simulink library "outp"  (R2021b)
(part 8 of 11)

      link override Signal_Override/_ovrdflg: Value=KOUTP_FDAGSCmd_enum_ovrdflg
      link override Signal_Override/_ovrdval: Value=KOUTP_FDAGSCmd_enum_ovrdval
  VTHC_FDBlowerCmd_pct_Inproc : FVT_lib/outp/OverrideAndLimit  SystemSampleTime=-1  VariantActivationTime=update diagram  Latency=0  AutoFrameSizeCalculation=off
      link override Signal_Limit/_maxval: Value=KOUTP_FDBlowerCmd_pct_maxval
      link override Signal_Limit/_minval: Value=KOUTP_FDBlowerCmd_pct_minval
      link override Signal_Override/_ovrdflg: Value=KOUTP_FDBlowerCmd_pct_ovrdflg
      link override Signal_Override/_ovrdval: Value=KOUTP_FDBlowerCmd_pct_ovrdval
  VTHC_FDCFGSAirIntCmd_enum_Inproc : FVT_lib/outp/OverrideAndLimit  SystemSampleTime=-1  VariantActivationTime=update diagram  Latency=0  AutoFrameSizeCalculation=off
      link override Signal_Limit/_maxval: Value=KOUTP_FDCFGSAirIntCmd_enum_maxval
      link override Signal_Limit/_minval: Value=KOUTP_FDCFGSAirIntCmd_enum_minval
      link override Signal_Override/_ovrdflg: Value=KOUTP_FDCFGSAirIntCmd_enum_ovrdflg
      link override Signal_Override/_ovrdval: Value=KOUTP_FDCFGSAirIntCmd_enum_ovrdval
  VTHC_FDCFGSAirIntStaSet123_enum_Inproc : FVT_lib/outp/OverrideAndLimit  SystemSampleTime=-1  VariantActivationTime=update diagram  Latency=0  AutoFrameSizeCalculation=off
      link override Signal_Limit/_maxval: Value=KOUTP_FDCFGSAirIntStaSet123_enum_maxval
      link override Signal_Limit/_minval: Value=KOUTP_FDCFGSAirIntStaSet123_enum_minval
      link override Signal_Override/_ovrdflg: Value=KOUTP_FDCFGSAirIntStaSet123_enum_ovrdflg
      link override Signal_Override/_ovrdval: Value=KOUTP_FDCFGSAirIntStaSet123_enum_ovrdval
  VTHC_FDCFGSAirIntStaSet457_enum_Inproc : FVT_lib/outp/OverrideAndLimit  SystemSampleTime=-1  VariantActivationTime=update diagram  Latency=0  AutoFrameSizeCalculation=off
      link override Signal_Limit/_maxval: Value=KOUTP_FDCFGSAirIntStaSet457_enum_maxval
      link override Signal_Limit/_minval: Value=KOUTP_FDCFGSAirIntStaSet457_enum_minval
      link override Signal_Override/_ovrdflg: Value=KOUTP_FDCFGSAirIntStaSet457_enum_ovrdflg
      link override Signal_Override/_ovrdval: Value=KOUTP_FDCFGSAirIntStaSet457_enum_ovrdval
  VTHC_FDCFGSAirIntSta_enum_Inproc : FVT_lib/outp/OverrideAndLimit  SystemSampleTime=-1  VariantActivationTime=update diagram  Latency=0  AutoFrameSizeCalculation=off
      link override Signal_Limit/_maxval: Value=KOUTP_FDCFGSAirIntSta_enum_maxval
      link override Signal_Limit/_minval: Value=KOUTP_FDCFGSAirIntSta_enum_minval
      link override Signal_Override/_ovrdflg: Value=KOUTP_FDCFGSAirIntSta_enum_ovrdflg
      link override Signal_Override/_ovrdval: Value=KOUTP_FDCFGSAirIntSta_enum_ovrdval
  VTHC_FDCFGSChCmd_enum_Inproc : FVT_lib/outp/OverrideAndLimit  SystemSampleTime=-1  VariantActivationTime=update diagram  Latency=0  AutoFrameSizeCalculation=off
      link override Signal_Limit/_maxval: Value=KOUTP_FDCFGSChCmd_enum_maxval
      link override Signal_Limit/_minval: Value=KOUTP_FDCFGSChCmd_enum_minval
      link override Signal_Override/_ovrdflg: Value=KOUTP_FDCFGSChCmd_enum_ovrdflg
      link override Signal_Override/_ovrdval: Value=KOUTP_FDCFGSChCmd_enum_ovrdval
  VTHC_FDCFGSChStaSet123_enum_Inproc : FVT_lib/outp/OverrideAndLimit  SystemSampleTime=-1  VariantActivationTime=update diagram  Latency=0  AutoFrameSizeCalculation=off
      link override Signal_Limit/_maxval: Value=KOUTP_FDCFGSChStaSet123_enum_maxval
      link override Signal_Limit/_minval: Value=KOUTP_FDCFGSChStaSet123_enum_minval
      link override Signal_Override/_ovrdflg: Value=KOUTP_FDCFGSChStaSet123_enum_ovrdflg
      link override Signal_Override/_ovrdval: Value=KOUTP_FDCFGSChStaSet123_enum_ovrdval
  VTHC_FDCFGSChStaSet457_enum_Inproc : FVT_lib/outp/OverrideAndLimit  SystemSampleTime=-1  VariantActivationTime=update diagram  Latency=0  AutoFrameSizeCalculation=off
      link override Signal_Limit/_maxval: Value=KOUTP_FDCFGSChStaSet457_enum_maxval
      link override Signal_Limit/_minval: Value=KOUTP_FDCFGSChStaSet457_enum_minval
      link override Signal_Override/_ovrdflg: Value=KOUTP_FDCFGSChStaSet457_enum_ovrdflg
      link override Signal_Override/_ovrdval: Value=KOUTP_FDCFGSChStaSet457_enum_ovrdval
  VTHC_FDCFGSChSta_enum_Inproc : FVT_lib/outp/OverrideAndLimit  SystemSampleTime=-1  VariantActivationTime=update diagram  Latency=0  AutoFrameSizeCalculation=off
      link override Signal_Limit/_maxval: Value=KOUTP_FDCFGSChSta_enum_maxval
      link override Signal_Limit/_minval: Value=KOUTP_FDCFGSChSta_enum_minval
      link override Signal_Override/_ovrdflg: Value=KOUTP_FDCFGSChSta_enum_ovrdflg
      link override Signal_Override/_ovrdval: Value=KOUTP_FDCFGSChSta_enum_ovrdval
  VTHC_FDCFGSFuncSta_enum_Inproc : FVT_lib/outp/OverrideAndLimit  SystemSampleTime=-1  VariantActivationTime=update diagram  Latency=0  AutoFrameSizeCalculation=off
      link override Signal_Limit/_maxval: Value=KOUTP_FDCFGSFuncSta_enum_maxval
      link override Signal_Limit/_minval: Value=KOUTP_FDCFGSFuncSta_enum_minval
      link override Signal_Override/_ovrdflg: Value=KOUTP_FDCFGSFuncSta_enum_ovrdflg
      link override Signal_Override/_ovrdval: Value=KOUTP_FDCFGSFuncSta_enum_ovrdval
  VTHC_FDCFGSFuncSta_flg_Inproc : FVT_lib/outp/OverrideAndLimit  SystemSampleTime=-1  VariantActivationTime=update diagram  Latency=0  AutoFrameSizeCalculation=off
      link override Signal_Limit/_maxval: Value=KOUTP_FDCFGSFuncSta_flg_maxval
      link override Signal_Limit/_minval: Value=KOUTP_FDCFGSFuncSta_flg_minval
      link override Signal_Override/_ovrdflg: Value=KOUTP_FDCFGSFuncSta_flg_ovrdflg
      link override Signal_Override/_ovrdval: Value=KOUTP_FDCFGSFuncSta_flg_ovrdval
  VTHC_FDCFGSIONCmd_flg_Inproc : FVT_lib/outp/OverrideAndLimit  SystemSampleTime=-1  VariantActivationTime=update diagram  Latency=0  AutoFrameSizeCalculation=off
      link override Signal_Limit/_maxval: Value=KOUTP_FDCFGSIONCmd_flg_maxval
      link override Signal_Limit/_minval: Value=KOUTP_FDCFGSIONCmd_flg_minval
      link override Signal_Override/_ovrdflg: Value=KOUTP_FDCFGSIONCmd_flg_ovrdflg
      link override Signal_Override/_ovrdval: Value=KOUTP_FDCFGSIONCmd_flg_ovrdval
  VTHC_FDCFGSIONSWSta_flg_Inproc : FVT_lib/outp/OverrideAndLimit  SystemSampleTime=-1  VariantActivationTime=update diagram  Latency=0  AutoFrameSizeCalculation=off
      link override Signal_Limit/_maxval: Value=KOUTP_FDCFGSIONSWSta_flg_maxval
      link override Signal_Limit/_minval: Value=KOUTP_FDCFGSIONSWSta_flg_minval
      link override Signal_Override/_ovrdflg: Value=KOUTP_FDCFGSIONSWSta_flg_ovrdflg
      link override Signal_Override/_ovrdval: Value=KOUTP_FDCFGSIONSWSta_flg_ovrdval
  VTHC_FDCFGSLearnCmd_enum_Inproc : FVT_lib/outp/OverrideAndLimit  SystemSampleTime=-1  VariantActivationTime=update diagram  Latency=0  AutoFrameSizeCalculation=off
      link override Signal_Limit/_maxval: Value=KOUTP_FDCFGSLearnCmd_enum_maxval
      link override Signal_Limit/_minval: Value=KOUTP_FDCFGSLearnCmd_enum_minval
      link override Signal_Override/_ovrdflg: Value=KOUTP_FDCFGSLearnCmd_enum_ovrdflg
      link override Signal_Override/_ovrdval: Value=KOUTP_FDCFGSLearnCmd_enum_ovrdval
  VTHC_FDCTHCAirIntZ3Sta_enum_Inproc : FVT_lib/outp/OverrideAndLimit  SystemSampleTime=-1  VariantActivationTime=update diagram  Latency=0  AutoFrameSizeCalculation=off
      link override Signal_Limit/_maxval: Value=KOUTP_FDCTHCAirIntZ3Sta_enum_maxval
      link override Signal_Limit/_minval: Value=KOUTP_FDCTHCAirIntZ3Sta_enum_minval
      link override Signal_Override/_ovrdflg: Value=KOUTP_FDCTHCAirIntZ3Sta_enum_ovrdflg
      link override Signal_Override/_ovrdval: Value=KOUTP_FDCTHCAirIntZ3Sta_enum_ovrdval
  VTHC_FDCTHCCLEVentYStaSet1_enum_Inproc : FVT_lib/outp/OverrideAndLimit  SystemSampleTime=-1  VariantActivationTime=update diagram  Latency=0  AutoFrameSizeCalculation=off
      link override Signal_Limit/_maxval: Value=KOUTP_FDCTHCCLEVentYStaSet1_enum_maxval
      link override Signal_Limit/_minval: Value=KOUTP_FDCTHCCLEVentYStaSet1_enum_minval
      link override Signal_Override/_ovrdflg: Value=KOUTP_FDCTHCCLEVentYStaSet1_enum_ovrdflg
      link override Signal_Override/_ovrdval: Value=KOUTP_FDCTHCCLEVentYStaSet1_enum_ovrdval
  VTHC_FDCTHCCLEVentYStaSet2_enum_Inproc : FVT_lib/outp/OverrideAndLimit  SystemSampleTime=-1  VariantActivationTime=update diagram  Latency=0  AutoFrameSizeCalculation=off
      link override Signal_Limit/_maxval: Value=KOUTP_FDCTHCCLEVentYStaSet2_enum_maxval
      link override Signal_Limit/_minval: Value=KOUTP_FDCTHCCLEVentYStaSet2_enum_minval
      link override Signal_Override/_ovrdflg: Value=KOUTP_FDCTHCCLEVentYStaSet2_enum_ovrdflg
      link override Signal_Override/_ovrdval: Value=KOUTP_FDCTHCCLEVentYStaSet2_enum_ovrdval
  VTHC_FDCTHCCLEVentYStaSet3_enum_Inproc : FVT_lib/outp/OverrideAndLimit  SystemSampleTime=-1  VariantActivationTime=update diagram  Latency=0  AutoFrameSizeCalculation=off
      link override Signal_Limit/_maxval: Value=KOUTP_FDCTHCCLEVentYStaSet3_enum_maxval
      link override Signal_Limit/_minval: Value=KOUTP_FDCTHCCLEVentYStaSet3_enum_minval
      link override Signal_Override/_ovrdflg: Value=KOUTP_FDCTHCCLEVentYStaSet3_enum_ovrdflg
      link override Signal_Override/_ovrdval: Value=KOUTP_FDCTHCCLEVentYStaSet3_enum_ovrdval
  VTHC_FDCTHCCLEVentYStaSet4_enum_Inproc : FVT_lib/outp/OverrideAndLimit  SystemSampleTime=-1  VariantActivationTime=update diagram  Latency=0  AutoFrameSizeCalculation=off
      link override Signal_Limit/_maxval: Value=KOUTP_FDCTHCCLEVentYStaSet4_enum_maxval
      link override Signal_Limit/_minval: Value=KOUTP_FDCTHCCLEVentYStaSet4_enum_minval
      link override Signal_Override/_ovrdflg: Value=KOUTP_FDCTHCCLEVentYStaSet4_enum_ovrdflg
      link override Signal_Override/_ovrdval: Value=KOUTP_FDCTHCCLEVentYStaSet4_enum_ovrdval
  VTHC_FDCTHCCLEVentYStaSet5_enum_Inproc : FVT_lib/outp/OverrideAndLimit  SystemSampleTime=-1  VariantActivationTime=update diagram  Latency=0  AutoFrameSizeCalculation=off
      link override Signal_Limit/_maxval: Value=KOUTP_FDCTHCCLEVentYStaSet5_enum_maxval
      link override Signal_Limit/_minval: Value=KOUTP_FDCTHCCLEVentYStaSet5_enum_minval
      link override Signal_Override/_ovrdflg: Value=KOUTP_FDCTHCCLEVentYStaSet5_enum_ovrdflg
      link override Signal_Override/_ovrdval: Value=KOUTP_FDCTHCCLEVentYStaSet5_enum_ovrdval
  VTHC_FDCTHCCLEVentYStaSet7_enum_Inproc : FVT_lib/outp/OverrideAndLimit  SystemSampleTime=-1  VariantActivationTime=update diagram  Latency=0  AutoFrameSizeCalculation=off
      link override Signal_Limit/_maxval: Value=KOUTP_FDCTHCCLEVentYStaSet7_enum_maxval
      link override Signal_Limit/_minval: Value=KOUTP_FDCTHCCLEVentYStaSet7_enum_minval
      link override Signal_Override/_ovrdflg: Value=KOUTP_FDCTHCCLEVentYStaSet7_enum_ovrdflg
      link override Signal_Override/_ovrdval: Value=KOUTP_FDCTHCCLEVentYStaSet7_enum_ovrdval
  VTHC_FDCTHCCLEVentYSta_enum_Inproc : FVT_lib/outp/OverrideAndLimit  SystemSampleTime=-1  VariantActivationTime=update diagram  Latency=0  AutoFrameSizeCalculation=off
      link override Signal_Limit/_maxval: Value=KOUTP_FDCTHCCLEVentYSta_enum_maxval
      link override Signal_Limit/_minval: Value=KOUTP_FDCTHCCLEVentYSta_enum_minval
      link override Signal_Override/_ovrdflg: Value=KOUTP_FDCTHCCLEVentYSta_enum_ovrdflg
      link override Signal_Override/_ovrdval: Value=KOUTP_FDCTHCCLEVentYSta_enum_ovrdval
  VTHC_FDCTHCCLEVentZStaSet1_enum_Inproc : FVT_lib/outp/OverrideAndLimit  SystemSampleTime=-1  VariantActivationTime=update diagram  Latency=0  AutoFrameSizeCalculation=off
      link override Signal_Limit/_maxval: Value=KOUTP_FDCTHCCLEVentZStaSet1_enum_maxval
      link override Signal_Limit/_minval: Value=KOUTP_FDCTHCCLEVentZStaSet1_enum_minval
      link override Signal_Override/_ovrdflg: Value=KOUTP_FDCTHCCLEVentZStaSet1_enum_ovrdflg
      link override Signal_Override/_ovrdval: Value=KOUTP_FDCTHCCLEVentZStaSet1_enum_ovrdval
  VTHC_FDCTHCCLEVentZStaSet2_enum_Inproc : FVT_lib/outp/OverrideAndLimit  SystemSampleTime=-1  VariantActivationTime=update diagram  Latency=0  AutoFrameSizeCalculation=off
      link override Signal_Limit/_maxval: Value=KOUTP_FDCTHCCLEVentZStaSet2_enum_maxval
      link override Signal_Limit/_minval: Value=KOUTP_FDCTHCCLEVentZStaSet2_enum_minval
      link override Signal_Override/_ovrdflg: Value=KOUTP_FDCTHCCLEVentZStaSet2_enum_ovrdflg
      link override Signal_Override/_ovrdval: Value=KOUTP_FDCTHCCLEVentZStaSet2_enum_ovrdval
  VTHC_FDCTHCCLEVentZStaSet3_enum_Inproc : FVT_lib/outp/OverrideAndLimit  SystemSampleTime=-1  VariantActivationTime=update diagram  Latency=0  AutoFrameSizeCalculation=off
      link override Signal_Limit/_maxval: Value=KOUTP_FDCTHCCLEVentZStaSet3_enum_maxval
      link override Signal_Limit/_minval: Value=KOUTP_FDCTHCCLEVentZStaSet3_enum_minval
      link override Signal_Override/_ovrdflg: Value=KOUTP_FDCTHCCLEVentZStaSet3_enum_ovrdflg
      link override Signal_Override/_ovrdval: Value=KOUTP_FDCTHCCLEVentZStaSet3_enum_ovrdval
  VTHC_FDCTHCCLEVentZStaSet4_enum_Inproc : FVT_lib/outp/OverrideAndLimit  SystemSampleTime=-1  VariantActivationTime=update diagram  Latency=0  AutoFrameSizeCalculation=off
      link override Signal_Limit/_maxval: Value=KOUTP_FDCTHCCLEVentZStaSet4_enum_maxval
      link override Signal_Limit/_minval: Value=KOUTP_FDCTHCCLEVentZStaSet4_enum_minval
      link override Signal_Override/_ovrdflg: Value=KOUTP_FDCTHCCLEVentZStaSet4_enum_ovrdflg
      link override Signal_Override/_ovrdval: Value=KOUTP_FDCTHCCLEVentZStaSet4_enum_ovrdval
  VTHC_FDCTHCCLEVentZStaSet5_enum_Inproc : FVT_lib/outp/OverrideAndLimit  SystemSampleTime=-1  VariantActivationTime=update diagram  Latency=0  AutoFrameSizeCalculation=off
      link override Signal_Limit/_maxval: Value=KOUTP_FDCTHCCLEVentZStaSet5_enum_maxval
      link override Signal_Limit/_minval: Value=KOUTP_FDCTHCCLEVentZStaSet5_enum_minval
      link override Signal_Override/_ovrdflg: Value=KOUTP_FDCTHCCLEVentZStaSet5_enum_ovrdflg
      link override Signal_Override/_ovrdval: Value=KOUTP_FDCTHCCLEVentZStaSet5_enum_ovrdval
  VTHC_FDCTHCCLEVentZStaSet7_enum_Inproc : FVT_lib/outp/OverrideAndLimit  SystemSampleTime=-1  VariantActivationTime=update diagram  Latency=0  AutoFrameSizeCalculation=off
      link override Signal_Limit/_maxval: Value=KOUTP_FDCTHCCLEVentZStaSet7_enum_maxval
      link override Signal_Limit/_minval: Value=KOUTP_FDCTHCCLEVentZStaSet7_enum_minval
      link override Signal_Override/_ovrdflg: Value=KOUTP_FDCTHCCLEVentZStaSet7_enum_ovrdflg
      link override Signal_Override/_ovrdval: Value=KOUTP_FDCTHCCLEVentZStaSet7_enum_ovrdval
  VTHC_FDCTHCCLEVentZSta_enum_Inproc : FVT_lib/outp/OverrideAndLimit  SystemSampleTime=-1  VariantActivationTime=update diagram  Latency=0  AutoFrameSizeCalculation=off
      link override Signal_Limit/_maxval: Value=KOUTP_FDCTHCCLEVentZSta_enum_maxval
      link override Signal_Limit/_minval: Value=KOUTP_FDCTHCCLEVentZSta_enum_minval
      link override Signal_Override/_ovrdflg: Value=KOUTP_FDCTHCCLEVentZSta_enum_ovrdflg
      link override Signal_Override/_ovrdval: Value=KOUTP_FDCTHCCLEVentZSta_enum_ovrdval
  VTHC_FDCTHCCLVentENSta_flg_Inproc : FVT_lib/outp/OverrideAndLimit  SystemSampleTime=-1  VariantActivationTime=update diagram  Latency=0  AutoFrameSizeCalculation=off
      link override Signal_Limit/_maxval: Value=KOUTP_FDCTHCCLVentENSta_flg_maxval
      link override Signal_Limit/_minval: Value=KOUTP_FDCTHCCLVentENSta_flg_minval
      link override Signal_Override/_ovrdflg: Value=KOUTP_FDCTHCCLVentENSta_flg_ovrdflg
      link override Signal_Override/_ovrdval: Value=KOUTP_FDCTHCCLVentENSta_flg_ovrdval
  VTHC_FDCTHCCREVentYStaSet1_enum_Inproc : FVT_lib/outp/OverrideAndLimit  SystemSampleTime=-1  VariantActivationTime=update diagram  Latency=0  AutoFrameSizeCalculation=off
      link override Signal_Limit/_maxval: Value=KOUTP_FDCTHCCREVentYStaSet1_enum_maxval
      link override Signal_Limit/_minval: Value=KOUTP_FDCTHCCREVentYStaSet1_enum_minval
      link override Signal_Override/_ovrdflg: Value=KOUTP_FDCTHCCREVentYStaSet1_enum_ovrdflg
      link override Signal_Override/_ovrdval: Value=KOUTP_FDCTHCCREVentYStaSet1_enum_ovrdval
  VTHC_FDCTHCCREVentYStaSet2_enum_Inproc : FVT_lib/outp/OverrideAndLimit  SystemSampleTime=-1  VariantActivationTime=update diagram  Latency=0  AutoFrameSizeCalculation=off
      link override Signal_Limit/_maxval: Value=KOUTP_FDCTHCCREVentYStaSet2_enum_maxval
      link override Signal_Limit/_minval: Value=KOUTP_FDCTHCCREVentYStaSet2_enum_minval
      link override Signal_Override/_ovrdflg: Value=KOUTP_FDCTHCCREVentYStaSet2_enum_ovrdflg
      link override Signal_Override/_ovrdval: Value=KOUTP_FDCTHCCREVentYStaSet2_enum_ovrdval
  VTHC_FDCTHCCREVentYStaSet3_enum_Inproc : FVT_lib/outp/OverrideAndLimit  SystemSampleTime=-1  VariantActivationTime=update diagram  Latency=0  AutoFrameSizeCalculation=off
      link override Signal_Limit/_maxval: Value=KOUTP_FDCTHCCREVentYStaSet3_enum_maxval
      link override Signal_Limit/_minval: Value=KOUTP_FDCTHCCREVentYStaSet3_enum_minval
      link override Signal_Override/_ovrdflg: Value=KOUTP_FDCTHCCREVentYStaSet3_enum_ovrdflg
      link override Signal_Override/_ovrdval: Value=KOUTP_FDCTHCCREVentYStaSet3_enum_ovrdval
  VTHC_FDCTHCCREVentYStaSet4_enum_Inproc : FVT_lib/outp/OverrideAndLimit  SystemSampleTime=-1  VariantActivationTime=update diagram  Latency=0  AutoFrameSizeCalculation=off
      link override Signal_Limit/_maxval: Value=KOUTP_FDCTHCCREVentYStaSet4_enum_maxval
      link override Signal_Limit/_minval: Value=KOUTP_FDCTHCCREVentYStaSet4_enum_minval
      link override Signal_Override/_ovrdflg: Value=KOUTP_FDCTHCCREVentYStaSet4_enum_ovrdflg
      link override Signal_Override/_ovrdval: Value=KOUTP_FDCTHCCREVentYStaSet4_enum_ovrdval
  VTHC_FDCTHCCREVentYStaSet5_enum_Inproc : FVT_lib/outp/OverrideAndLimit  SystemSampleTime=-1  VariantActivationTime=update diagram  Latency=0  AutoFrameSizeCalculation=off
      link override Signal_Limit/_maxval: Value=KOUTP_FDCTHCCREVentYStaSet5_enum_maxval
      link override Signal_Limit/_minval: Value=KOUTP_FDCTHCCREVentYStaSet5_enum_minval
      link override Signal_Override/_ovrdflg: Value=KOUTP_FDCTHCCREVentYStaSet5_enum_ovrdflg
      link override Signal_Override/_ovrdval: Value=KOUTP_FDCTHCCREVentYStaSet5_enum_ovrdval
  VTHC_FDCTHCCREVentYStaSet7_enum_Inproc : FVT_lib/outp/OverrideAndLimit  SystemSampleTime=-1  VariantActivationTime=update diagram  Latency=0  AutoFrameSizeCalculation=off
      link override Signal_Limit/_maxval: Value=KOUTP_FDCTHCCREVentYStaSet7_enum_maxval
      link override Signal_Limit/_minval: Value=KOUTP_FDCTHCCREVentYStaSet7_enum_minval
      link override Signal_Override/_ovrdflg: Value=KOUTP_FDCTHCCREVentYStaSet7_enum_ovrdflg
      link override Signal_Override/_ovrdval: Value=KOUTP_FDCTHCCREVentYStaSet7_enum_ovrdval
  VTHC_FDCTHCCREVentYSta_enum_Inproc : FVT_lib/outp/OverrideAndLimit  SystemSampleTime=-1  VariantActivationTime=update diagram  Latency=0  AutoFrameSizeCalculation=off
      link override Signal_Limit/_maxval: Value=KOUTP_FDCTHCCREVentYSta_enum_maxval
      link override Signal_Limit/_minval: Value=KOUTP_FDCTHCCREVentYSta_enum_minval
      link override Signal_Override/_ovrdflg: Value=KOUTP_FDCTHCCREVentYSta_enum_ovrdflg
      link override Signal_Override/_ovrdval: Value=KOUTP_FDCTHCCREVentYSta_enum_ovrdval
  VTHC_FDCTHCCREVentZStaSet1_enum_Inproc : FVT_lib/outp/OverrideAndLimit  SystemSampleTime=-1  VariantActivationTime=update diagram  Latency=0  AutoFrameSizeCalculation=off
      link override Signal_Limit/_maxval: Value=KOUTP_FDCTHCCREVentZStaSet1_enum_maxval
      link override Signal_Limit/_minval: Value=KOUTP_FDCTHCCREVentZStaSet1_enum_minval
      link override Signal_Override/_ovrdflg: Value=KOUTP_FDCTHCCREVentZStaSet1_enum_ovrdflg
      link override Signal_Override/_ovrdval: Value=KOUTP_FDCTHCCREVentZStaSet1_enum_ovrdval
  VTHC_FDCTHCCREVentZStaSet2_enum_Inproc : FVT_lib/outp/OverrideAndLimit  SystemSampleTime=-1  VariantActivationTime=update diagram  Latency=0  AutoFrameSizeCalculation=off
      link override Signal_Limit/_maxval: Value=KOUTP_FDCTHCCREVentZStaSet2_enum_maxval
      link override Signal_Limit/_minval: Value=KOUTP_FDCTHCCREVentZStaSet2_enum_minval
      link override Signal_Override/_ovrdflg: Value=KOUTP_FDCTHCCREVentZStaSet2_enum_ovrdflg
      link override Signal_Override/_ovrdval: Value=KOUTP_FDCTHCCREVentZStaSet2_enum_ovrdval
  VTHC_FDCTHCCREVentZStaSet3_enum_Inproc : FVT_lib/outp/OverrideAndLimit  SystemSampleTime=-1  VariantActivationTime=update diagram  Latency=0  AutoFrameSizeCalculation=off
      link override Signal_Limit/_maxval: Value=KOUTP_FDCTHCCREVentZStaSet3_enum_maxval
      link override Signal_Limit/_minval: Value=KOUTP_FDCTHCCREVentZStaSet3_enum_minval
      link override Signal_Override/_ovrdflg: Value=KOUTP_FDCTHCCREVentZStaSet3_enum_ovrdflg
      link override Signal_Override/_ovrdval: Value=KOUTP_FDCTHCCREVentZStaSet3_enum_ovrdval
  VTHC_FDCTHCCREVentZStaSet4_enum_Inproc : FVT_lib/outp/OverrideAndLimit  SystemSampleTime=-1  VariantActivationTime=update diagram  Latency=0  AutoFrameSizeCalculation=off
      link override Signal_Limit/_maxval: Value=KOUTP_FDCTHCCREVentZStaSet4_enum_maxval
      link override Signal_Limit/_minval: Value=KOUTP_FDCTHCCREVentZStaSet4_enum_minval
      link override Signal_Override/_ovrdflg: Value=KOUTP_FDCTHCCREVentZStaSet4_enum_ovrdflg
      link override Signal_Override/_ovrdval: Value=KOUTP_FDCTHCCREVentZStaSet4_enum_ovrdval
  VTHC_FDCTHCCREVentZStaSet5_enum_Inproc : FVT_lib/outp/OverrideAndLimit  SystemSampleTime=-1  VariantActivationTime=update diagram  Latency=0  AutoFrameSizeCalculation=off
      link override Signal_Limit/_maxval: Value=KOUTP_FDCTHCCREVentZStaSet5_enum_maxval
      link override Signal_Limit/_minval: Value=KOUTP_FDCTHCCREVentZStaSet5_enum_minval
      link override Signal_Override/_ovrdflg: Value=KOUTP_FDCTHCCREVentZStaSet5_enum_ovrdflg
      link override Signal_Override/_ovrdval: Value=KOUTP_FDCTHCCREVentZStaSet5_enum_ovrdval
  VTHC_FDCTHCCREVentZStaSet7_enum_Inproc : FVT_lib/outp/OverrideAndLimit  SystemSampleTime=-1  VariantActivationTime=update diagram  Latency=0  AutoFrameSizeCalculation=off
      link override Signal_Limit/_maxval: Value=KOUTP_FDCTHCCREVentZStaSet7_enum_maxval
      link override Signal_Limit/_minval: Value=KOUTP_FDCTHCCREVentZStaSet7_enum_minval
      link override Signal_Override/_ovrdflg: Value=KOUTP_FDCTHCCREVentZStaSet7_enum_ovrdflg
      link override Signal_Override/_ovrdval: Value=KOUTP_FDCTHCCREVentZStaSet7_enum_ovrdval
  VTHC_FDCTHCCREVentZSta_enum_Inproc : FVT_lib/outp/OverrideAndLimit  SystemSampleTime=-1  VariantActivationTime=update diagram  Latency=0  AutoFrameSizeCalculation=off
      link override Signal_Limit/_maxval: Value=KOUTP_FDCTHCCREVentZSta_enum_maxval
      link override Signal_Limit/_minval: Value=KOUTP_FDCTHCCREVentZSta_enum_minval
      link override Signal_Override/_ovrdflg: Value=KOUTP_FDCTHCCREVentZSta_enum_ovrdflg
      link override Signal_Override/_ovrdval: Value=KOUTP_FDCTHCCREVentZSta_enum_ovrdval
  VTHC_FDCTHCCRVentENSta_flg_Inproc : FVT_lib/outp/OverrideAndLimit  SystemSampleTime=-1  VariantActivationTime=update diagram  Latency=0  AutoFrameSizeCalculation=off
      link override Signal_Limit/_maxval: Value=KOUTP_FDCTHCCRVentENSta_flg_maxval
      link override Signal_Limit/_minval: Value=KOUTP_FDCTHCCRVentENSta_flg_minval
      link override Signal_Override/_ovrdflg: Value=KOUTP_FDCTHCCRVentENSta_flg_ovrdflg
      link override Signal_Override/_ovrdval: Value=KOUTP_FDCTHCCRVentENSta_flg_ovrdval
  VTHC_FDCTHCLEVentModeSta_enum_Inproc : FVT_lib/outp/OverrideAndLimit  SystemSampleTime=-1  VariantActivationTime=update diagram  Latency=0  AutoFrameSizeCalculation=off
      link override Signal_Limit/_maxval: Value=KOUTP_FDCTHCLEVentModeSta_enum_maxval
      link override Signal_Limit/_minval: Value=KOUTP_FDCTHCLEVentModeSta_enum_minval
      link override Signal_Override/_ovrdflg: Value=KOUTP_FDCTHCLEVentModeSta_enum_ovrdflg
      link override Signal_Override/_ovrdval: Value=KOUTP_FDCTHCLEVentModeSta_enum_ovrdval
  VTHC_FDCTHCLEVentYStaSet1_enum_Inproc : FVT_lib/outp/OverrideAndLimit  SystemSampleTime=-1  VariantActivationTime=update diagram  Latency=0  AutoFrameSizeCalculation=off
      link override Signal_Limit/_maxval: Value=KOUTP_FDCTHCLEVentYStaSet1_enum_maxval
      link override Signal_Limit/_minval: Value=KOUTP_FDCTHCLEVentYStaSet1_enum_minval
      link override Signal_Override/_ovrdflg: Value=KOUTP_FDCTHCLEVentYStaSet1_enum_ovrdflg
      link override Signal_Override/_ovrdval: Value=KOUTP_FDCTHCLEVentYStaSet1_enum_ovrdval
  VTHC_FDCTHCLEVentYStaSet2_enum_Inproc : FVT_lib/outp/OverrideAndLimit  SystemSampleTime=-1  VariantActivationTime=update diagram  Latency=0  AutoFrameSizeCalculation=off
      link override Signal_Limit/_maxval: Value=KOUTP_FDCTHCLEVentYStaSet2_enum_maxval
      link override Signal_Limit/_minval: Value=KOUTP_FDCTHCLEVentYStaSet2_enum_minval
      link override Signal_Override/_ovrdflg: Value=KOUTP_FDCTHCLEVentYStaSet2_enum_ovrdflg
      link override Signal_Override/_ovrdval: Value=KOUTP_FDCTHCLEVentYStaSet2_enum_ovrdval
  VTHC_FDCTHCLEVentYStaSet3_enum_Inproc : FVT_lib/outp/OverrideAndLimit  SystemSampleTime=-1  VariantActivationTime=update diagram  Latency=0  AutoFrameSizeCalculation=off
      link override Signal_Limit/_maxval: Value=KOUTP_FDCTHCLEVentYStaSet3_enum_maxval
      link override Signal_Limit/_minval: Value=KOUTP_FDCTHCLEVentYStaSet3_enum_minval
      link override Signal_Override/_ovrdflg: Value=KOUTP_FDCTHCLEVentYStaSet3_enum_ovrdflg
      link override Signal_Override/_ovrdval: Value=KOUTP_FDCTHCLEVentYStaSet3_enum_ovrdval
  VTHC_FDCTHCLEVentYStaSet4_enum_Inproc : FVT_lib/outp/OverrideAndLimit  SystemSampleTime=-1  VariantActivationTime=update diagram  Latency=0  AutoFrameSizeCalculation=off
      link override Signal_Limit/_maxval: Value=KOUTP_FDCTHCLEVentYStaSet4_enum_maxval
      link override Signal_Limit/_minval: Value=KOUTP_FDCTHCLEVentYStaSet4_enum_minval
      link override Signal_Override/_ovrdflg: Value=KOUTP_FDCTHCLEVentYStaSet4_enum_ovrdflg
      link override Signal_Override/_ovrdval: Value=KOUTP_FDCTHCLEVentYStaSet4_enum_ovrdval
  VTHC_FDCTHCLEVentYStaSet5_enum_Inproc : FVT_lib/outp/OverrideAndLimit  SystemSampleTime=-1  VariantActivationTime=update diagram  Latency=0  AutoFrameSizeCalculation=off
      link override Signal_Limit/_maxval: Value=KOUTP_FDCTHCLEVentYStaSet5_enum_maxval
      link override Signal_Limit/_minval: Value=KOUTP_FDCTHCLEVentYStaSet5_enum_minval
      link override Signal_Override/_ovrdflg: Value=KOUTP_FDCTHCLEVentYStaSet5_enum_ovrdflg
      link override Signal_Override/_ovrdval: Value=KOUTP_FDCTHCLEVentYStaSet5_enum_ovrdval
  VTHC_FDCTHCLEVentYStaSet7_enum_Inproc : FVT_lib/outp/OverrideAndLimit  SystemSampleTime=-1  VariantActivationTime=update diagram  Latency=0  AutoFrameSizeCalculation=off
      link override Signal_Limit/_maxval: Value=KOUTP_FDCTHCLEVentYStaSet7_enum_maxval
      link override Signal_Limit/_minval: Value=KOUTP_FDCTHCLEVentYStaSet7_enum_minval
      link override Signal_Override/_ovrdflg: Value=KOUTP_FDCTHCLEVentYStaSet7_enum_ovrdflg
      link override Signal_Override/_ovrdval: Value=KOUTP_FDCTHCLEVentYStaSet7_enum_ovrdval
  VTHC_FDCTHCLEVentYSta_enum_Inproc : FVT_lib/outp/OverrideAndLimit  SystemSampleTime=-1  VariantActivationTime=update diagram  Latency=0  AutoFrameSizeCalculation=off
      link override Signal_Limit/_maxval: Value=KOUTP_FDCTHCLEVentYSta_enum_maxval
      link override Signal_Limit/_minval: Value=KOUTP_FDCTHCLEVentYSta_enum_minval
      link override Signal_Override/_ovrdflg: Value=KOUTP_FDCTHCLEVentYSta_enum_ovrdflg
      link override Signal_Override/_ovrdval: Value=KOUTP_FDCTHCLEVentYSta_enum_ovrdval
  VTHC_FDCTHCLEVentZStaSet1_enum_Inproc : FVT_lib/outp/OverrideAndLimit  SystemSampleTime=-1  VariantActivationTime=update diagram  Latency=0  AutoFrameSizeCalculation=off
      link override Signal_Limit/_maxval: Value=KOUTP_FDCTHCLEVentZStaSet1_enum_maxval
      link override Signal_Limit/_minval: Value=KOUTP_FDCTHCLEVentZStaSet1_enum_minval
      link override Signal_Override/_ovrdflg: Value=KOUTP_FDCTHCLEVentZStaSet1_enum_ovrdflg
      link override Signal_Override/_ovrdval: Value=KOUTP_FDCTHCLEVentZStaSet1_enum_ovrdval
  VTHC_FDCTHCLEVentZStaSet2_enum_Inproc : FVT_lib/outp/OverrideAndLimit  SystemSampleTime=-1  VariantActivationTime=update diagram  Latency=0  AutoFrameSizeCalculation=off
      link override Signal_Limit/_maxval: Value=KOUTP_FDCTHCLEVentZStaSet2_enum_maxval
      link override Signal_Limit/_minval: Value=KOUTP_FDCTHCLEVentZStaSet2_enum_minval
      link override Signal_Override/_ovrdflg: Value=KOUTP_FDCTHCLEVentZStaSet2_enum_ovrdflg
      link override Signal_Override/_ovrdval: Value=KOUTP_FDCTHCLEVentZStaSet2_enum_ovrdval
  VTHC_FDCTHCLEVentZStaSet3_enum_Inproc : FVT_lib/outp/OverrideAndLimit  SystemSampleTime=-1  VariantActivationTime=update diagram  Latency=0  AutoFrameSizeCalculation=off
      link override Signal_Limit/_maxval: Value=KOUTP_FDCTHCLEVentZStaSet3_enum_maxval
      link override Signal_Limit/_minval: Value=KOUTP_FDCTHCLEVentZStaSet3_enum_minval
      link override Signal_Override/_ovrdflg: Value=KOUTP_FDCTHCLEVentZStaSet3_enum_ovrdflg
      link override Signal_Override/_ovrdval: Value=KOUTP_FDCTHCLEVentZStaSet3_enum_ovrdval
  VTHC_FDCTHCLEVentZStaSet4_enum_Inproc : FVT_lib/outp/OverrideAndLimit  SystemSampleTime=-1  VariantActivationTime=update diagram  Latency=0  AutoFrameSizeCalculation=off
      link override Signal_Limit/_maxval: Value=KOUTP_FDCTHCLEVentZStaSet4_enum_maxval
      link override Signal_Limit/_minval: Value=KOUTP_FDCTHCLEVentZStaSet4_enum_minval
      link override Signal_Override/_ovrdflg: Value=KOUTP_FDCTHCLEVentZStaSet4_enum_ovrdflg
      link override Signal_Override/_ovrdval: Value=KOUTP_FDCTHCLEVentZStaSet4_enum_ovrdval
  VTHC_FDCTHCLEVentZStaSet5_enum_Inproc : FVT_lib/outp/OverrideAndLimit  SystemSampleTime=-1  VariantActivationTime=update diagram  Latency=0  AutoFrameSizeCalculation=off
      link override Signal_Limit/_maxval: Value=KOUTP_FDCTHCLEVentZStaSet5_enum_maxval
      link override Signal_Limit/_minval: Value=KOUTP_FDCTHCLEVentZStaSet5_enum_minval
      link override Signal_Override/_ovrdflg: Value=KOUTP_FDCTHCLEVentZStaSet5_enum_ovrdflg
      link override Signal_Override/_ovrdval: Value=KOUTP_FDCTHCLEVentZStaSet5_enum_ovrdval
  VTHC_FDCTHCLEVentZStaSet7_enum_Inproc : FVT_lib/outp/OverrideAndLimit  SystemSampleTime=-1  VariantActivationTime=update diagram  Latency=0  AutoFrameSizeCalculation=off
      link override Signal_Limit/_maxval: Value=KOUTP_FDCTHCLEVentZStaSet7_enum_maxval
      link override Signal_Limit/_minval: Value=KOUTP_FDCTHCLEVentZStaSet7_enum_minval
      link override Signal_Override/_ovrdflg: Value=KOUTP_FDCTHCLEVentZStaSet7_enum_ovrdflg
      link override Signal_Override/_ovrdval: Value=KOUTP_FDCTHCLEVentZStaSet7_enum_ovrdval
  VTHC_FDCTHCLEVentZSta_enum_Inproc : FVT_lib/outp/OverrideAndLimit  SystemSampleTime=-1  VariantActivationTime=update diagram  Latency=0  AutoFrameSizeCalculation=off
      link override Signal_Limit/_maxval: Value=KOUTP_FDCTHCLEVentZSta_enum_maxval
      link override Signal_Limit/_minval: Value=KOUTP_FDCTHCLEVentZSta_enum_minval
      link override Signal_Override/_ovrdflg: Value=KOUTP_FDCTHCLEVentZSta_enum_ovrdflg
      link override Signal_Override/_ovrdval: Value=KOUTP_FDCTHCLEVentZSta_enum_ovrdval
  VTHC_FDCTHCLVentENSta_flg_Inproc : FVT_lib/outp/OverrideAndLimit  SystemSampleTime=-1  VariantActivationTime=update diagram  Latency=0  AutoFrameSizeCalculation=off
      link override Signal_Limit/_maxval: Value=KOUTP_FDCTHCLVentENSta_flg_maxval
      link override Signal_Limit/_minval: Value=KOUTP_FDCTHCLVentENSta_flg_minval
      link override Signal_Override/_ovrdflg: Value=KOUTP_FDCTHCLVentENSta_flg_ovrdflg
      link override Signal_Override/_ovrdval: Value=KOUTP_FDCTHCLVentENSta_flg_ovrdval
  VTHC_FDCTHCMAPTCForceOFFSta_flg_Inproc : FVT_lib/outp/OverrideAndLimit  SystemSampleTime=-1  VariantActivationTime=update diagram  Latency=0  AutoFrameSizeCalculation=off
      link override Signal_Limit/_maxval: Value=KOUTP_FDCTHCMAPTCForceOFFSta_flg_maxval
      link override Signal_Limit/_minval: Value=KOUTP_FDCTHCMAPTCForceOFFSta_flg_minval
      link override Signal_Override/_ovrdflg: Value=KOUTP_FDCTHCMAPTCForceOFFSta_flg_ovrdflg
      link override Signal_Override/_ovrdval: Value=KOUTP_FDCTHCMAPTCForceOFFSta_flg_ovrdval
  VTHC_FDCTHCMPreWPTCHeatSta_enum_Inproc : FVT_lib/outp/OverrideAndLimit  SystemSampleTime=-1  VariantActivationTime=update diagram  Latency=0  AutoFrameSizeCalculation=off
      link override Signal_Limit/_maxval: Value=KOUTP_FDCTHCMPreWPTCHeatSta_enum_maxval
      link override Signal_Limit/_minval: Value=KOUTP_FDCTHCMPreWPTCHeatSta_enum_minval
      link override Signal_Override/_ovrdflg: Value=KOUTP_FDCTHCMPreWPTCHeatSta_enum_ovrdflg
      link override Signal_Override/_ovrdval: Value=KOUTP_FDCTHCMPreWPTCHeatSta_enum_ovrdval
  VTHC_FDCTHCREVentModeSta_enum_Inproc : FVT_lib/outp/OverrideAndLimit  SystemSampleTime=-1  VariantActivationTime=update diagram  Latency=0  AutoFrameSizeCalculation=off
      link override Signal_Limit/_maxval: Value=KOUTP_FDCTHCREVentModeSta_enum_maxval
      link override Signal_Limit/_minval: Value=KOUTP_FDCTHCREVentModeSta_enum_minval
      link override Signal_Override/_ovrdflg: Value=KOUTP_FDCTHCREVentModeSta_enum_ovrdflg
      link override Signal_Override/_ovrdval: Value=KOUTP_FDCTHCREVentModeSta_enum_ovrdval
  VTHC_FDCTHCREVentYStaSet1_enum_Inproc : FVT_lib/outp/OverrideAndLimit  SystemSampleTime=-1  VariantActivationTime=update diagram  Latency=0  AutoFrameSizeCalculation=off
      link override Signal_Limit/_maxval: Value=KOUTP_FDCTHCREVentYStaSet1_enum_maxval
      link override Signal_Limit/_minval: Value=KOUTP_FDCTHCREVentYStaSet1_enum_minval
      link override Signal_Override/_ovrdflg: Value=KOUTP_FDCTHCREVentYStaSet1_enum_ovrdflg
      link override Signal_Override/_ovrdval: Value=KOUTP_FDCTHCREVentYStaSet1_enum_ovrdval
  VTHC_FDCTHCREVentYStaSet2_enum_Inproc : FVT_lib/outp/OverrideAndLimit  SystemSampleTime=-1  VariantActivationTime=update diagram  Latency=0  AutoFrameSizeCalculation=off
      link override Signal_Limit/_maxval: Value=KOUTP_FDCTHCREVentYStaSet2_enum_maxval
      link override Signal_Limit/_minval: Value=KOUTP_FDCTHCREVentYStaSet2_enum_minval
      link override Signal_Override/_ovrdflg: Value=KOUTP_FDCTHCREVentYStaSet2_enum_ovrdflg
      link override Signal_Override/_ovrdval: Value=KOUTP_FDCTHCREVentYStaSet2_enum_ovrdval
  VTHC_FDCTHCREVentYStaSet3_enum_Inproc : FVT_lib/outp/OverrideAndLimit  SystemSampleTime=-1  VariantActivationTime=update diagram  Latency=0  AutoFrameSizeCalculation=off
      link override Signal_Limit/_maxval: Value=KOUTP_FDCTHCREVentYStaSet3_enum_maxval
      link override Signal_Limit/_minval: Value=KOUTP_FDCTHCREVentYStaSet3_enum_minval
      link override Signal_Override/_ovrdflg: Value=KOUTP_FDCTHCREVentYStaSet3_enum_ovrdflg
      link override Signal_Override/_ovrdval: Value=KOUTP_FDCTHCREVentYStaSet3_enum_ovrdval
  VTHC_FDCTHCREVentYStaSet4_enum_Inproc : FVT_lib/outp/OverrideAndLimit  SystemSampleTime=-1  VariantActivationTime=update diagram  Latency=0  AutoFrameSizeCalculation=off
      link override Signal_Limit/_maxval: Value=KOUTP_FDCTHCREVentYStaSet4_enum_maxval
      link override Signal_Limit/_minval: Value=KOUTP_FDCTHCREVentYStaSet4_enum_minval
      link override Signal_Override/_ovrdflg: Value=KOUTP_FDCTHCREVentYStaSet4_enum_ovrdflg
      link override Signal_Override/_ovrdval: Value=KOUTP_FDCTHCREVentYStaSet4_enum_ovrdval
  VTHC_FDCTHCREVentYStaSet5_enum_Inproc : FVT_lib/outp/OverrideAndLimit  SystemSampleTime=-1  VariantActivationTime=update diagram  Latency=0  AutoFrameSizeCalculation=off
      link override Signal_Limit/_maxval: Value=KOUTP_FDCTHCREVentYStaSet5_enum_maxval
      link override Signal_Limit/_minval: Value=KOUTP_FDCTHCREVentYStaSet5_enum_minval
      link override Signal_Override/_ovrdflg: Value=KOUTP_FDCTHCREVentYStaSet5_enum_ovrdflg
      link override Signal_Override/_ovrdval: Value=KOUTP_FDCTHCREVentYStaSet5_enum_ovrdval
  VTHC_FDCTHCREVentYStaSet7_enum_Inproc : FVT_lib/outp/OverrideAndLimit  SystemSampleTime=-1  VariantActivationTime=update diagram  Latency=0  AutoFrameSizeCalculation=off
      link override Signal_Limit/_maxval: Value=KOUTP_FDCTHCREVentYStaSet7_enum_maxval
      link override Signal_Limit/_minval: Value=KOUTP_FDCTHCREVentYStaSet7_enum_minval
      link override Signal_Override/_ovrdflg: Value=KOUTP_FDCTHCREVentYStaSet7_enum_ovrdflg
      link override Signal_Override/_ovrdval: Value=KOUTP_FDCTHCREVentYStaSet7_enum_ovrdval
  VTHC_FDCTHCREVentYSta_enum_Inproc : FVT_lib/outp/OverrideAndLimit  SystemSampleTime=-1  VariantActivationTime=update diagram  Latency=0  AutoFrameSizeCalculation=off
      link override Signal_Limit/_maxval: Value=KOUTP_FDCTHCREVentYSta_enum_maxval
      link override Signal_Limit/_minval: Value=KOUTP_FDCTHCREVentYSta_enum_minval
      link override Signal_Override/_ovrdflg: Value=KOUTP_FDCTHCREVentYSta_enum_ovrdflg
      link override Signal_Override/_ovrdval: Value=KOUTP_FDCTHCREVentYSta_enum_ovrdval
  VTHC_FDCTHCREVentZStaSet1_enum_Inproc : FVT_lib/outp/OverrideAndLimit  SystemSampleTime=-1  VariantActivationTime=update diagram  Latency=0  AutoFrameSizeCalculation=off
      link override Signal_Limit/_maxval: Value=KOUTP_FDCTHCREVentZStaSet1_enum_maxval
      link override Signal_Limit/_minval: Value=KOUTP_FDCTHCREVentZStaSet1_enum_minval
      link override Signal_Override/_ovrdflg: Value=KOUTP_FDCTHCREVentZStaSet1_enum_ovrdflg
      link override Signal_Override/_ovrdval: Value=KOUTP_FDCTHCREVentZStaSet1_enum_ovrdval
  VTHC_FDCTHCREVentZStaSet2_enum_Inproc : FVT_lib/outp/OverrideAndLimit  SystemSampleTime=-1  VariantActivationTime=update diagram  Latency=0  AutoFrameSizeCalculation=off
      link override Signal_Limit/_maxval: Value=KOUTP_FDCTHCREVentZStaSet2_enum_maxval
      link override Signal_Limit/_minval: Value=KOUTP_FDCTHCREVentZStaSet2_enum_minval
      link override Signal_Override/_ovrdflg: Value=KOUTP_FDCTHCREVentZStaSet2_enum_ovrdflg
      link override Signal_Override/_ovrdval: Value=KOUTP_FDCTHCREVentZStaSet2_enum_ovrdval
  VTHC_FDCTHCREVentZStaSet3_enum_Inproc : FVT_lib/outp/OverrideAndLimit  SystemSampleTime=-1  VariantActivationTime=update diagram  Latency=0  AutoFrameSizeCalculation=off
      link override Signal_Limit/_maxval: Value=KOUTP_FDCTHCREVentZStaSet3_enum_maxval
      link override Signal_Limit/_minval: Value=KOUTP_FDCTHCREVentZStaSet3_enum_minval
      link override Signal_Override/_ovrdflg: Value=KOUTP_FDCTHCREVentZStaSet3_enum_ovrdflg
      link override Signal_Override/_ovrdval: Value=KOUTP_FDCTHCREVentZStaSet3_enum_ovrdval
  VTHC_FDCTHCREVentZStaSet4_enum_Inproc : FVT_lib/outp/OverrideAndLimit  SystemSampleTime=-1  VariantActivationTime=update diagram  Latency=0  AutoFrameSizeCalculation=off
      link override Signal_Limit/_maxval: Value=KOUTP_FDCTHCREVentZStaSet4_enum_maxval
      link override Signal_Limit/_minval: Value=KOUTP_FDCTHCREVentZStaSet4_enum_minval
      link override Signal_Override/_ovrdflg: Value=KOUTP_FDCTHCREVentZStaSet4_enum_ovrdflg
      link override Signal_Override/_ovrdval: Value=KOUTP_FDCTHCREVentZStaSet4_enum_ovrdval
  VTHC_FDCTHCREVentZStaSet5_enum_Inproc : FVT_lib/outp/OverrideAndLimit  SystemSampleTime=-1  VariantActivationTime=update diagram  Latency=0  AutoFrameSizeCalculation=off
      link override Signal_Limit/_maxval: Value=KOUTP_FDCTHCREVentZStaSet5_enum_maxval
      link override Signal_Limit/_minval: Value=KOUTP_FDCTHCREVentZStaSet5_enum_minval
      link override Signal_Override/_ovrdflg: Value=KOUTP_FDCTHCREVentZStaSet5_enum_ovrdflg
      link override Signal_Override/_ovrdval: Value=KOUTP_FDCTHCREVentZStaSet5_enum_ovrdval
  VTHC_FDCTHCREVentZStaSet7_enum_Inproc : FVT_lib/outp/OverrideAndLimit  SystemSampleTime=-1  VariantActivationTime=update diagram  Latency=0  AutoFrameSizeCalculation=off
      link override Signal_Limit/_maxval: Value=KOUTP_FDCTHCREVentZStaSet7_enum_maxval
      link override Signal_Limit/_minval: Value=KOUTP_FDCTHCREVentZStaSet7_enum_minval
      link override Signal_Override/_ovrdflg: Value=KOUTP_FDCTHCREVentZStaSet7_enum_ovrdflg
      link override Signal_Override/_ovrdval: Value=KOUTP_FDCTHCREVentZStaSet7_enum_ovrdval
  VTHC_FDCTHCREVentZSta_enum_Inproc : FVT_lib/outp/OverrideAndLimit  SystemSampleTime=-1  VariantActivationTime=update diagram  Latency=0  AutoFrameSizeCalculation=off
      link override Signal_Limit/_maxval: Value=KOUTP_FDCTHCREVentZSta_enum_maxval
      link override Signal_Limit/_minval: Value=KOUTP_FDCTHCREVentZSta_enum_minval
      link override Signal_Override/_ovrdflg: Value=KOUTP_FDCTHCREVentZSta_enum_ovrdflg
      link override Signal_Override/_ovrdval: Value=KOUTP_FDCTHCREVentZSta_enum_ovrdval
  VTHC_FDCTHCRVentENSta_flg_Inproc : FVT_lib/outp/OverrideAndLimit  SystemSampleTime=-1  VariantActivationTime=update diagram  Latency=0  AutoFrameSizeCalculation=off
      link override Signal_Limit/_maxval: Value=KOUTP_FDCTHCRVentENSta_flg_maxval
      link override Signal_Limit/_minval: Value=KOUTP_FDCTHCRVentENSta_flg_minval
      link override Signal_Override/_ovrdflg: Value=KOUTP_FDCTHCRVentENSta_flg_ovrdflg
      link override Signal_Override/_ovrdval: Value=KOUTP_FDCTHCRVentENSta_flg_ovrdval
  VTHC_FDCompCmd_rpm_Inproc : FVT_lib/outp/OverrideAndLimit  SystemSampleTime=-1  VariantActivationTime=update diagram  Latency=0  AutoFrameSizeCalculation=off
      link override Signal_Limit/_maxval: Value=KOUTP_FDCompCmd_rpm_maxval
      link override Signal_Limit/_minval: Value=KOUTP_FDCompCmd_rpm_minval
      link override Signal_Override/_ovrdflg: Value=KOUTP_FDCompCmd_rpm_ovrdflg
      link override Signal_Override/_ovrdval: Value=KOUTP_FDCompCmd_rpm_ovrdval
  VTHC_FDEWP1Cmd_enum_Inproc : FVT_lib/outp/OverrideAndLimit  SystemSampleTime=-1  VariantActivationTime=update diagram  Latency=0  AutoFrameSizeCalculation=off
      link override Signal_Limit/_maxval: Value=KOUTP_FDEWP1Cmd_enum_maxval
      link override Signal_Limit/_minval: Value=KOUTP_FDEWP1Cmd_enum_minval
      link override Signal_Override/_ovrdflg: Value=KOUTP_FDEWP1Cmd_enum_ovrdflg
      link override Signal_Override/_ovrdval: Value=KOUTP_FDEWP1Cmd_enum_ovrdval
  VTHC_FDEWP2Cmd_enum_Inproc : FVT_lib/outp/OverrideAndLimit  SystemSampleTime=-1  VariantActivationTime=update diagram  Latency=0  AutoFrameSizeCalculation=off
      link override Signal_Limit/_maxval: Value=KOUTP_FDEWP2Cmd_enum_maxval
      link override Signal_Limit/_minval: Value=KOUTP_FDEWP2Cmd_enum_minval
      link override Signal_Override/_ovrdflg: Value=KOUTP_FDEWP2Cmd_enum_ovrdflg
      link override Signal_Override/_ovrdval: Value=KOUTP_FDEWP2Cmd_enum_ovrdval
  VTHC_FDEWP3Cmd_enum_Inproc : FVT_lib/outp/OverrideAndLimit  SystemSampleTime=-1  VariantActivationTime=update diagram  Latency=0  AutoFrameSizeCalculation=off
      link override Signal_Limit/_maxval: Value=KOUTP_FDEWP3Cmd_enum_maxval
      link override Signal_Limit/_minval: Value=KOUTP_FDEWP3Cmd_enum_minval
      link override Signal_Override/_ovrdflg: Value=KOUTP_FDEWP3Cmd_enum_ovrdflg
      link override Signal_Override/_ovrdval: Value=KOUTP_FDEWP3Cmd_enum_ovrdval
  VTHC_FDEXV1Cmd_step_Inproc : FVT_lib/outp/OverrideAndLimit  SystemSampleTime=-1  VariantActivationTime=update diagram  Latency=0  AutoFrameSizeCalculation=off
      link override Signal_Limit/_maxval: Value=KOUTP_FDEXV1Cmd_step_maxval
      link override Signal_Limit/_minval: Value=KOUTP_FDEXV1Cmd_step_minval
      link override Signal_Override/_ovrdflg: Value=KOUTP_FDEXV1Cmd_step_ovrdflg
      link override Signal_Override/_ovrdval: Value=KOUTP_FDEXV1Cmd_step_ovrdval
  VTHC_FDEXV2Cmd_step_Inproc : FVT_lib/outp/OverrideAndLimit  SystemSampleTime=-1  VariantActivationTime=update diagram  Latency=0  AutoFrameSizeCalculation=off
      link override Signal_Limit/_maxval: Value=KOUTP_FDEXV2Cmd_step_maxval
      link override Signal_Limit/_minval: Value=KOUTP_FDEXV2Cmd_step_minval
      link override Signal_Override/_ovrdflg: Value=KOUTP_FDEXV2Cmd_step_ovrdflg
      link override Signal_Override/_ovrdval: Value=KOUTP_FDEXV2Cmd_step_ovrdval
  VTHC_FDFWVCmd_flg_Inproc : FVT_lib/outp/OverrideAndLimit  SystemSampleTime=-1  VariantActivationTime=update diagram  Latency=0  AutoFrameSizeCalculation=off
      link override Signal_Limit/_maxval: Value=KOUTP_FDFWVCmd_flg_maxval
      link override Signal_Limit/_minval: Value=KOUTP_FDFWVCmd_flg_minval
      link override Signal_Override/_ovrdflg: Value=KOUTP_FDFWVCmd_flg_ovrdflg
      link override Signal_Override/_ovrdval: Value=KOUTP_FDFWVCmd_flg_ovrdval
  VTHC_FDFrLeAPTCHeatPwrCmd_W_Inproc : FVT_lib/outp/OverrideAndLimit  SystemSampleTime=-1  VariantActivationTime=update diagram  Latency=0  AutoFrameSizeCalculation=off
      link override Signal_Limit/_maxval: Value=KOUTP_FDFrLeAPTCHeatPwrCmd_W_maxval
      link override Signal_Limit/_minval: Value=KOUTP_FDFrLeAPTCHeatPwrCmd_W_minval
      link override Signal_Override/_ovrdflg: Value=KOUTP_FDFrLeAPTCHeatPwrCmd_W_ovrdflg
      link override Signal_Override/_ovrdval: Value=KOUTP_FDFrLeAPTCHeatPwrCmd_W_ovrdval
  VTHC_FDFrRiAPTCHeatPwrCmd_W_Inproc : FVT_lib/outp/OverrideAndLimit  SystemSampleTime=-1  VariantActivationTime=update diagram  Latency=0  AutoFrameSizeCalculation=off
      link override Signal_Limit/_maxval: Value=KOUTP_FDFrRiAPTCHeatPwrCmd_W_maxval
      link override Signal_Limit/_minval: Value=KOUTP_FDFrRiAPTCHeatPwrCmd_W_minval
      link override Signal_Override/_ovrdflg: Value=KOUTP_FDFrRiAPTCHeatPwrCmd_W_ovrdflg
      link override Signal_Override/_ovrdval: Value=KOUTP_FDFrRiAPTCHeatPwrCmd_W_ovrdval
  VTHC_FDFrWPTCHeatPwrCmd_W_Inproc : FVT_lib/outp/OverrideAndLimit  SystemSampleTime=-1  VariantActivationTime=update diagram  Latency=0  AutoFrameSizeCalculation=off
      link override Signal_Limit/_maxval: Value=KOUTP_FDFrWPTCHeatPwrCmd_W_maxval
      link override Signal_Limit/_minval: Value=KOUTP_FDFrWPTCHeatPwrCmd_W_minval
      link override Signal_Override/_ovrdflg: Value=KOUTP_FDFrWPTCHeatPwrCmd_W_ovrdflg
      link override Signal_Override/_ovrdval: Value=KOUTP_FDFrWPTCHeatPwrCmd_W_ovrdval
  VTHC_FDRecyAutoCmd_enum_Inproc : FVT_lib/outp/OverrideAndLimit  SystemSampleTime=-1  VariantActivationTime=update diagram  Latency=0  AutoFrameSizeCalculation=off
      link override Signal_Limit/_maxval: Value=KOUTP_FDRecyAutoCmd_enum_maxval
      link override Signal_Limit/_minval: Value=KOUTP_FDRecyAutoCmd_enum_minval
      link override Signal_Override/_ovrdflg: Value=KOUTP_FDRecyAutoCmd_enum_ovrdflg
      link override Signal_Override/_ovrdval: Value=KOUTP_FDRecyAutoCmd_enum_ovrdval
  VTHC_FDRrAPTCHeatPwrCmd_W_Inproc : FVT_lib/outp/OverrideAndLimit  SystemSampleTime=-1  VariantActivationTime=update diagram  Latency=0  AutoFrameSizeCalculation=off
      link override Signal_Limit/_maxval: Value=KOUTP_FDRrAPTCHeatPwrCmd_W_maxval
      link override Signal_Limit/_minval: Value=KOUTP_FDRrAPTCHeatPwrCmd_W_minval
      link override Signal_Override/_ovrdflg: Value=KOUTP_FDRrAPTCHeatPwrCmd_W_ovrdflg
      link override Signal_Override/_ovrdval: Value=KOUTP_FDRrAPTCHeatPwrCmd_W_ovrdval
  VTHC_FDSOTXVCmd_flg_Inproc : FVT_lib/outp/OverrideAndLimit  SystemSampleTime=-1  VariantActivationTime=update diagram  Latency=0  AutoFrameSizeCalculation=off
      link override Signal_Limit/_maxval: Value=KOUTP_FDSOTXVCmd_flg_maxval
      link override Signal_Limit/_minval: Value=KOUTP_FDSOTXVCmd_flg_minval
      link override Signal_Override/_ovrdflg: Value=KOUTP_FDSOTXVCmd_flg_ovrdflg
      link override Signal_Override/_ovrdval: Value=KOUTP_FDSOTXVCmd_flg_ovrdval
  VTHC_FDSOV1Cmd_flg_Inproc : FVT_lib/outp/OverrideAndLimit  SystemSampleTime=-1  VariantActivationTime=update diagram  Latency=0  AutoFrameSizeCalculation=off
      link override Signal_Limit/_maxval: Value=KOUTP_FDSOV1Cmd_flg_maxval
      link override Signal_Limit/_minval: Value=KOUTP_FDSOV1Cmd_flg_minval
      link override Signal_Override/_ovrdflg: Value=KOUTP_FDSOV1Cmd_flg_ovrdflg
      link override Signal_Override/_ovrdval: Value=KOUTP_FDSOV1Cmd_flg_ovrdval
  VTHC_FDSOV2Cmd_flg_Inproc : FVT_lib/outp/OverrideAndLimit  SystemSampleTime=-1  VariantActivationTime=update diagram  Latency=0  AutoFrameSizeCalculation=off
      link override Signal_Limit/_maxval: Value=KOUTP_FDSOV2Cmd_flg_maxval
      link override Signal_Limit/_minval: Value=KOUTP_FDSOV2Cmd_flg_minval
      link override Signal_Override/_ovrdflg: Value=KOUTP_FDSOV2Cmd_flg_ovrdflg
      link override Signal_Override/_ovrdval: Value=KOUTP_FDSOV2Cmd_flg_ovrdval
  VTHC_FDSOV3Cmd_flg_Inproc : FVT_lib/outp/OverrideAndLimit  SystemSampleTime=-1  VariantActivationTime=update diagram  Latency=0  AutoFrameSizeCalculation=off
      link override Signal_Limit/_maxval: Value=KOUTP_FDSOV3Cmd_flg_maxval
      link override Signal_Limit/_minval: Value=KOUTP_FDSOV3Cmd_flg_minval
      link override Signal_Override/_ovrdflg: Value=KOUTP_FDSOV3Cmd_flg_ovrdflg
      link override Signal_Override/_ovrdval: Value=KOUTP_FDSOV3Cmd_flg_ovrdval
  VTHC_FDTWVCmd_pct_Inproc : FVT_lib/outp/OverrideAndLimit  SystemSampleTime=-1  VariantActivationTime=update diagram  Latency=0  AutoFrameSizeCalculation=off
      link override Signal_Limit/_maxval: Value=KOUTP_FDTWVCmd_pct_maxval
      link override Signal_Limit/_minval: Value=KOUTP_FDTWVCmd_pct_minval
      link override Signal_Override/_ovrdflg: Value=KOUTP_FDTWVCmd_pct_ovrdflg
      link override Signal_Override/_ovrdval: Value=KOUTP_FDTWVCmd_pct_ovrdval
  VTHC_FOOTSet_enum_Inproc : FVT_lib/outp/OverrideAndLimit  SystemSampleTime=-1  VariantActivationTime=update diagram  Latency=0  AutoFrameSizeCalculation=off
      link override Signal_Limit/_maxval: Value=KOUTP_FOOTSet_enum_maxval
      link override Signal_Limit/_minval: Value=KOUTP_FOOTSet_enum_minval
      link override Signal_Override/_ovrdflg: Value=KOUTP_FOOTSet_enum_ovrdflg
      link override Signal_Override/_ovrdval: Value=KOUTP_FOOTSet_enum_ovrdval
  VTHC_FaceMSet_enum_Inproc : FVT_lib/outp/OverrideAndLimit  SystemSampleTime=-1  VariantActivationTime=update diagram  Latency=0  AutoFrameSizeCalculation=off
      link override Signal_Limit/_maxval: Value=KOUTP_FaceMSet_enum_maxval
      link override Signal_Limit/_minval: Value=KOUTP_FaceMSet_enum_minval
      link override Signal_Override/_ovrdflg: Value=KOUTP_FaceMSet_enum_ovrdflg
      link override Signal_Override/_ovrdval: Value=KOUTP_FaceMSet_enum_ovrdval
  VTHC_FaceM_flg_Inproc : FVT_lib/outp/OverrideAndLimit  SystemSampleTime=-1  VariantActivationTime=update diagram  Latency=0  AutoFrameSizeCalculation=off
      link override Signal_Limit/_maxval: Value=KOUTP_FaceM_flg_maxval
      link override Signal_Limit/_minval: Value=KOUTP_FaceM_flg_minval
      link override Signal_Override/_ovrdflg: Value=KOUTP_FaceM_flg_ovrdflg
      link override Signal_Override/_ovrdval: Value=KOUTP_FaceM_flg_ovrdval
  VTHC_Face_flg_Inproc : FVT_lib/outp/OverrideAndLimit  SystemSampleTime=-1  VariantActivationTime=update diagram  Latency=0  AutoFrameSizeCalculation=off
      link override Signal_Limit/_maxval: Value=KOUTP_Face_flg_maxval
      link override Signal_Limit/_minval: Value=KOUTP_Face_flg_minval
      link override Signal_Override/_ovrdflg: Value=KOUTP_Face_flg_ovrdflg
      link override Signal_Override/_ovrdval: Value=KOUTP_Face_flg_ovrdval
  VTHC_FootMSet_enum_Inproc : FVT_lib/outp/OverrideAndLimit  SystemSampleTime=-1  VariantActivationTime=update diagram  Latency=0  AutoFrameSizeCalculation=off
      link override Signal_Limit/_maxval: Value=KOUTP_FootMSet_enum_maxval
      link override Signal_Limit/_minval: Value=KOUTP_FootMSet_enum_minval
      link override Signal_Override/_ovrdflg: Value=KOUTP_FootMSet_enum_ovrdflg
      link override Signal_Override/_ovrdval: Value=KOUTP_FootMSet_enum_ovrdval
  VTHC_FootM_flg_Inproc : FVT_lib/outp/OverrideAndLimit  SystemSampleTime=-1  VariantActivationTime=update diagram  Latency=0  AutoFrameSizeCalculation=off
      link override Signal_Limit/_maxval: Value=KOUTP_FootM_flg_maxval
      link override Signal_Limit/_minval: Value=KOUTP_FootM_flg_minval
      link override Signal_Override/_ovrdflg: Value=KOUTP_FootM_flg_ovrdflg
      link override Signal_Override/_ovrdval: Value=KOUTP_FootM_flg_ovrdval
  VTHC_Foot_flg_Inproc : FVT_lib/outp/OverrideAndLimit  SystemSampleTime=-1  VariantActivationTime=update diagram  Latency=0  AutoFrameSizeCalculation=off
      link override Signal_Limit/_maxval: Value=KOUTP_Foot_flg_maxval
      link override Signal_Limit/_minval: Value=KOUTP_Foot_flg_minval
      link override Signal_Override/_ovrdflg: Value=KOUTP_Foot_flg_ovrdflg
      link override Signal_Override/_ovrdval: Value=KOUTP_Foot_flg_ovrdval
  VTHC_FrostSet_enum_Inproc : FVT_lib/outp/OverrideAndLimit  SystemSampleTime=-1  VariantActivationTime=update diagram  Latency=0  AutoFrameSizeCalculation=off
      link override Signal_Limit/_maxval: Value=KOUTP_FrostSet_enum_maxval
      link override Signal_Limit/_minval: Value=KOUTP_FrostSet_enum_minval
      link override Signal_Override/_ovrdflg: Value=KOUTP_FrostSet_enum_ovrdflg
      link override Signal_Override/_ovrdval: Value=KOUTP_FrostSet_enum_ovrdval
  VTHC_Frost_flg_Inproc : FVT_lib/outp/OverrideAndLimit  SystemSampleTime=-1  VariantActivationTime=update diagram  Latency=0  AutoFrameSizeCalculation=off
      link override Signal_Limit/_maxval: Value=KOUTP_Frost_flg_maxval
      link override Signal_Limit/_minval: Value=KOUTP_Frost_flg_minval
      link override Signal_Override/_ovrdflg: Value=KOUTP_Frost_flg_ovrdflg
      link override Signal_Override/_ovrdval: Value=KOUTP_Frost_flg_ovrdval
  VTHC_IONSWStaSet_enum_Inproc : FVT_lib/outp/OverrideAndLimit  SystemSampleTime=-1  VariantActivationTime=update diagram  Latency=0  AutoFrameSizeCalculation=off
      link override Signal_Limit/_maxval: Value=KOUTP_IONSWStaSet_enum_maxval
      link override Signal_Limit/_minval: Value=KOUTP_IONSWStaSet_enum_minval
      link override Signal_Override/_ovrdflg: Value=KOUTP_IONSWStaSet_enum_ovrdflg
      link override Signal_Override/_ovrdval: Value=KOUTP_IONSWStaSet_enum_ovrdval
  VTHC_LEVentModeStaSet123_enum_Inproc : FVT_lib/outp/OverrideAndLimit  SystemSampleTime=-1  VariantActivationTime=update diagram  Latency=0  AutoFrameSizeCalculation=off
      link override Signal_Limit/_maxval: Value=KOUTP_LEVentModeStaSet123_enum_maxval
      link override Signal_Limit/_minval: Value=KOUTP_LEVentModeStaSet123_enum_minval
      link override Signal_Override/_ovrdflg: Value=KOUTP_LEVentModeStaSet123_enum_ovrdflg
      link override Signal_Override/_ovrdval: Value=KOUTP_LEVentModeStaSet123_enum_ovrdval
  VTHC_LEVentModeStaSet457_enum_Inproc : FVT_lib/outp/OverrideAndLimit  SystemSampleTime=-1  VariantActivationTime=update diagram  Latency=0  AutoFrameSizeCalculation=off
      link override Signal_Limit/_maxval: Value=KOUTP_LEVentModeStaSet457_enum_maxval
      link override Signal_Limit/_minval: Value=KOUTP_LEVentModeStaSet457_enum_minval
      link override Signal_Override/_ovrdflg: Value=KOUTP_LEVentModeStaSet457_enum_ovrdflg
      link override Signal_Override/_ovrdval: Value=KOUTP_LEVentModeStaSet457_enum_ovrdval
  VTHC_LVentENSet_enum_Inproc : FVT_lib/outp/OverrideAndLimit  SystemSampleTime=-1  VariantActivationTime=update diagram  Latency=0  AutoFrameSizeCalculation=off
      link override Signal_Limit/_maxval: Value=KOUTP_LVentENSet_enum_maxval
      link override Signal_Limit/_minval: Value=KOUTP_LVentENSet_enum_minval
      link override Signal_Override/_ovrdflg: Value=KOUTP_LVentENSet_enum_ovrdflg
      link override Signal_Override/_ovrdval: Value=KOUTP_LVentENSet_enum_ovrdval
  VTHC_LVentEN_flg_Inproc : FVT_lib/outp/OverrideAndLimit  SystemSampleTime=-1  VariantActivationTime=update diagram  Latency=0  AutoFrameSizeCalculation=off
      link override Signal_Limit/_maxval: Value=KOUTP_LVentEN_flg_maxval
      link override Signal_Limit/_minval: Value=KOUTP_LVentEN_flg_minval
      link override Signal_Override/_ovrdflg: Value=KOUTP_LVentEN_flg_ovrdflg
      link override Signal_Override/_ovrdval: Value=KOUTP_LVentEN_flg_ovrdval
  VTHC_REVentModeStaSet123_enum_Inproc : FVT_lib/outp/OverrideAndLimit  SystemSampleTime=-1  VariantActivationTime=update diagram  Latency=0  AutoFrameSizeCalculation=off
      link override Signal_Limit/_maxval: Value=KOUTP_REVentModeStaSet123_enum_maxval
      link override Signal_Limit/_minval: Value=KOUTP_REVentModeStaSet123_enum_minval
      link override Signal_Override/_ovrdflg: Value=KOUTP_REVentModeStaSet123_enum_ovrdflg
      link override Signal_Override/_ovrdval: Value=KOUTP_REVentModeStaSet123_enum_ovrdval
  VTHC_REVentModeStaSet457_enum_Inproc : FVT_lib/outp/OverrideAndLimit  SystemSampleTime=-1  VariantActivationTime=update diagram  Latency=0  AutoFrameSizeCalculation=off
      link override Signal_Limit/_maxval: Value=KOUTP_REVentModeStaSet457_enum_maxval
      link override Signal_Limit/_minval: Value=KOUTP_REVentModeStaSet457_enum_minval
      link override Signal_Override/_ovrdflg: Value=KOUTP_REVentModeStaSet457_enum_ovrdflg
      link override Signal_Override/_ovrdval: Value=KOUTP_REVentModeStaSet457_enum_ovrdval
  VTHC_RVentENSet_enum_Inproc : FVT_lib/outp/OverrideAndLimit  SystemSampleTime=-1  VariantActivationTime=update diagram  Latency=0  AutoFrameSizeCalculation=off
      link override Signal_Limit/_maxval: Value=KOUTP_RVentENSet_enum_maxval
      link override Signal_Limit/_minval: Value=KOUTP_RVentENSet_enum_minval
      link override Signal_Override/_ovrdflg: Value=KOUTP_RVentENSet_enum_ovrdflg
      link override Signal_Override/_ovrdval: Value=KOUTP_RVentENSet_enum_ovrdval
  VTHC_RVentEN_flg_Inproc : FVT_lib/outp/OverrideAndLimit  SystemSampleTime=-1  VariantActivationTime=update diagram  Latency=0  AutoFrameSizeCalculation=off
      link override Signal_Limit/_maxval: Value=KOUTP_RVentEN_flg_maxval
      link override Signal_Limit/_minval: Value=KOUTP_RVentEN_flg_minval
      link override Signal_Override/_ovrdflg: Value=KOUTP_RVentEN_flg_ovrdflg
      link override Signal_Override/_ovrdval: Value=KOUTP_RVentEN_flg_ovrdval
  VTHC_RecAutoFlg_flg_Inproc : FVT_lib/outp/OverrideAndLimit  SystemSampleTime=-1  VariantActivationTime=update diagram  Latency=0  AutoFrameSizeCalculation=off
      link override Signal_Limit/_maxval: Value=KOUTP_RecAutoFlg_flg_maxval
      link override Signal_Limit/_minval: Value=KOUTP_RecAutoFlg_flg_minval
      link override Signal_Override/_ovrdflg: Value=KOUTP_RecAutoFlg_flg_ovrdflg
      link override Signal_Override/_ovrdval: Value=KOUTP_RecAutoFlg_flg_ovrdval
  VTHC_RecyAutoSet_enum_Inproc : FVT_lib/outp/OverrideAndLimit  SystemSampleTime=-1  VariantActivationTime=update diagram  Latency=0  AutoFrameSizeCalculation=off
      link override Signal_Limit/_maxval: Value=KOUTP_RecyAutoSet_enum_maxval
      link override Signal_Limit/_minval: Value=KOUTP_RecyAutoSet_enum_minval
      link override Signal_Override/_ovrdflg: Value=KOUTP_RecyAutoSet_enum_ovrdflg
      link override Signal_Override/_ovrdval: Value=KOUTP_RecyAutoSet_enum_ovrdval
  VTHC_SettempZon1Set1_enum_Inproc : FVT_lib/outp/OverrideAndLimit  SystemSampleTime=-1  VariantActivationTime=update diagram  Latency=0  AutoFrameSizeCalculation=off
      link override Signal_Limit/_maxval: Value=KOUTP_SettempZon1Set1_enum_maxval
      link override Signal_Limit/_minval: Value=KOUTP_SettempZon1Set1_enum_minval
      link override Signal_Override/_ovrdflg: Value=KOUTP_SettempZon1Set1_enum_ovrdflg
      link override Signal_Override/_ovrdval: Value=KOUTP_SettempZon1Set1_enum_ovrdval
  VTHC_SettempZon1Set2_enum_Inproc : FVT_lib/outp/OverrideAndLimit  SystemSampleTime=-1  VariantActivationTime=update diagram  Latency=0  AutoFrameSizeCalculation=off
      link override Signal_Limit/_maxval: Value=KOUTP_SettempZon1Set2_enum_maxval
      link override Signal_Limit/_minval: Value=KOUTP_SettempZon1Set2_enum_minval
      link override Signal_Override/_ovrdflg: Value=KOUTP_SettempZon1Set2_enum_ovrdflg
      link override Signal_Override/_ovrdval: Value=KOUTP_SettempZon1Set2_enum_ovrdval
  VTHC_SettempZon1Set3_enum_Inproc : FVT_lib/outp/OverrideAndLimit  SystemSampleTime=-1  VariantActivationTime=update diagram  Latency=0  AutoFrameSizeCalculation=off
      link override Signal_Limit/_maxval: Value=KOUTP_SettempZon1Set3_enum_maxval
      link override Signal_Limit/_minval: Value=KOUTP_SettempZon1Set3_enum_minval
      link override Signal_Override/_ovrdflg: Value=KOUTP_SettempZon1Set3_enum_ovrdflg
      link override Signal_Override/_ovrdval: Value=KOUTP_SettempZon1Set3_enum_ovrdval
  VTHC_SettempZon1Set4_enum_Inproc : FVT_lib/outp/OverrideAndLimit  SystemSampleTime=-1  VariantActivationTime=update diagram  Latency=0  AutoFrameSizeCalculation=off
      link override Signal_Limit/_maxval: Value=KOUTP_SettempZon1Set4_enum_maxval
      link override Signal_Limit/_minval: Value=KOUTP_SettempZon1Set4_enum_minval
      link override Signal_Override/_ovrdflg: Value=KOUTP_SettempZon1Set4_enum_ovrdflg
      link override Signal_Override/_ovrdval: Value=KOUTP_SettempZon1Set4_enum_ovrdval
  VTHC_SettempZon1Set5_enum_Inproc : FVT_lib/outp/OverrideAndLimit  SystemSampleTime=-1  VariantActivationTime=update diagram  Latency=0  AutoFrameSizeCalculation=off
      link override Signal_Limit/_maxval: Value=KOUTP_SettempZon1Set5_enum_maxval
      link override Signal_Limit/_minval: Value=KOUTP_SettempZon1Set5_enum_minval
      link override Signal_Override/_ovrdflg: Value=KOUTP_SettempZon1Set5_enum_ovrdflg
      link override Signal_Override/_ovrdval: Value=KOUTP_SettempZon1Set5_enum_ovrdval
  VTHC_SettempZon1Set7_enum_Inproc : FVT_lib/outp/OverrideAndLimit  SystemSampleTime=-1  VariantActivationTime=update diagram  Latency=0  AutoFrameSizeCalculation=off
      link override Signal_Limit/_maxval: Value=KOUTP_SettempZon1Set7_enum_maxval
      link override Signal_Limit/_minval: Value=KOUTP_SettempZon1Set7_enum_minval
      link override Signal_Override/_ovrdflg: Value=KOUTP_SettempZon1Set7_enum_ovrdflg
      link override Signal_Override/_ovrdval: Value=KOUTP_SettempZon1Set7_enum_ovrdval
  VTHC_THSysErrlampReq_flg_Inproc : FVT_lib/outp/OverrideAndLimit  SystemSampleTime=-1  VariantActivationTime=update diagram  Latency=0  AutoFrameSizeCalculation=off
      link override Signal_Limit/_maxval: Value=KOUTP_THSysErrlampReq_flg_maxval
      link override Signal_Limit/_minval: Value=KOUTP_THSysErrlampReq_flg_minval
      link override Signal_Override/_ovrdflg: Value=KOUTP_THSysErrlampReq_flg_ovrdflg
      link override Signal_Override/_ovrdval: Value=KOUTP_THSysErrlampReq_flg_ovrdval
  VTHC_fdefogSet_enum_Inproc : FVT_lib/outp/OverrideAndLimit  SystemSampleTime=-1  VariantActivationTime=update diagram  Latency=0  AutoFrameSizeCalculation=off
      link override Signal_Limit/_maxval: Value=KOUTP_fdefogSet_enum_maxval
      link override Signal_Limit/_minval: Value=KOUTP_fdefogSet_enum_minval
      link override Signal_Override/_ovrdflg: Value=KOUTP_fdefogSet_enum_ovrdflg
      link override Signal_Override/_ovrdval: Value=KOUTP_fdefogSet_enum_ovrdval
  VTHC_fdefog_flg_Inproc : FVT_lib/outp/OverrideAndLimit  SystemSampleTime=-1  VariantActivationTime=update diagram  Latency=0  AutoFrameSizeCalculation=off
      link override Signal_Limit/_maxval: Value=KOUTP_fdefog_flg_maxval
      link override Signal_Limit/_minval: Value=KOUTP_fdefog_flg_minval
      link override Signal_Override/_ovrdflg: Value=KOUTP_fdefog_flg_ovrdflg
      link override Signal_Override/_ovrdval: Value=KOUTP_fdefog_flg_ovrdval
  VTHC_sigAirIntenZon1St_enum_Inproc : FVT_lib/outp/OverrideAndLimit  SystemSampleTime=-1  VariantActivationTime=update diagram  Latency=0  AutoFrameSizeCalculation=off
      link override Signal_Limit/_maxval: Value=KOUTP_sigAirIntenZon1St_enum_maxval
      link override Signal_Limit/_minval: Value=KOUTP_sigAirIntenZon1St_enum_minval
      link override Signal_Override/_ovrdflg: Value=KOUTP_sigAirIntenZon1St_enum_ovrdflg
      link override Signal_Override/_ovrdval: Value=KOUTP_sigAirIntenZon1St_enum_ovrdval
  VTHC_sigAmbAirT_C_Inproc : FVT_lib/outp/OverrideAndLimit  SystemSampleTime=-1  VariantActivationTime=update diagram  Latency=0  AutoFrameSizeCalculation=off
      link override Signal_Limit/_maxval: Value=KOUTP_sigAmbAirT_C_maxval
      link override Signal_Limit/_minval: Value=KOUTP_sigAmbAirT_C_minval
      link override Signal_Override/_ovrdflg: Value=KOUTP_sigAmbAirT_C_ovrdflg
      link override Signal_Override/_ovrdval: Value=KOUTP_sigAmbAirT_C_ovrdval
  VTHC_sigCbnAirT_C_Inproc : FVT_lib/outp/OverrideAndLimit  SystemSampleTime=-1  VariantActivationTime=update diagram  Latency=0  AutoFrameSizeCalculation=off
      link override Signal_Limit/_maxval: Value=KOUTP_sigCbnAirT_C_maxval
      link override Signal_Limit/_minval: Value=KOUTP_sigCbnAirT_C_minval
      link override Signal_Override/_ovrdflg: Value=KOUTP_sigCbnAirT_C_ovrdflg
      link override Signal_Override/_ovrdval: Value=KOUTP_sigCbnAirT_C_ovrdval
  VTHC_sigCbnSolarLeft_W_Inproc : FVT_lib/outp/OverrideAndLimit  SystemSampleTime=-1  VariantActivationTime=update diagram  Latency=0  AutoFrameSizeCalculation=off
      link override Signal_Limit/_maxval: Value=KOUTP_sigCbnSolarLeft_W_maxval
      link override Signal_Limit/_minval: Value=KOUTP_sigCbnSolarLeft_W_minval
      link override Signal_Override/_ovrdflg: Value=KOUTP_sigCbnSolarLeft_W_ovrdflg
      link override Signal_Override/_ovrdval: Value=KOUTP_sigCbnSolarLeft_W_ovrdval
  VTHC_sigCbnSolarRight_W_Inproc : FVT_lib/outp/OverrideAndLimit  SystemSampleTime=-1  VariantActivationTime=update diagram  Latency=0  AutoFrameSizeCalculation=off
      link override Signal_Limit/_maxval: Value=KOUTP_sigCbnSolarRight_W_maxval
      link override Signal_Limit/_minval: Value=KOUTP_sigCbnSolarRight_W_minval
      link override Signal_Override/_ovrdflg: Value=KOUTP_sigCbnSolarRight_W_ovrdflg
      link override Signal_Override/_ovrdval: Value=KOUTP_sigCbnSolarRight_W_ovrdval
  VTHC_sigClntTHvBattIn_C_Inproc : FVT_lib/outp/OverrideAndLimit  SystemSampleTime=-1  VariantActivationTime=update diagram  Latency=0  AutoFrameSizeCalculation=off
      link override Signal_Limit/_maxval: Value=KOUTP_sigClntTHvBattIn_C_maxval
      link override Signal_Limit/_minval: Value=KOUTP_sigClntTHvBattIn_C_minval
      link override Signal_Override/_ovrdflg: Value=KOUTP_sigClntTHvBattIn_C_ovrdflg
      link override Signal_Override/_ovrdval: Value=KOUTP_sigClntTHvBattIn_C_ovrdval
  VTHC_sigClntTHvBattOut_C_Inproc : FVT_lib/outp/OverrideAndLimit  SystemSampleTime=-1  VariantActivationTime=update diagram  Latency=0  AutoFrameSizeCalculation=off
      link override Signal_Limit/_maxval: Value=KOUTP_sigClntTHvBattOut_C_maxval
      link override Signal_Limit/_minval: Value=KOUTP_sigClntTHvBattOut_C_minval
      link override Signal_Override/_ovrdflg: Value=KOUTP_sigClntTHvBattOut_C_ovrdflg
      link override Signal_Override/_ovrdval: Value=KOUTP_sigClntTHvBattOut_C_ovrdval
  VTHC_sigDfrstSt_flg_Inproc : FVT_lib/outp/OverrideAndLimit  SystemSampleTime=-1  VariantActivationTime=update diagram  Latency=0  AutoFrameSizeCalculation=off
      link override Signal_Limit/_maxval: Value=KOUTP_sigDfrstSt_flg_maxval
      link override Signal_Limit/_minval: Value=KOUTP_sigDfrstSt_flg_minval
      link override Signal_Override/_ovrdflg: Value=KOUTP_sigDfrstSt_flg_ovrdflg
      link override Signal_Override/_ovrdval: Value=KOUTP_sigDfrstSt_flg_ovrdval
  VTHC_sigRecircStSet_enum_Inproc : FVT_lib/outp/OverrideAndLimit  SystemSampleTime=-1  VariantActivationTime=update diagram  Latency=0  AutoFrameSizeCalculation=off
      link override Signal_Limit/_maxval: Value=KOUTP_sigRecircStSet_enum_maxval
      link override Signal_Limit/_minval: Value=KOUTP_sigRecircStSet_enum_minval
      link override Signal_Override/_ovrdflg: Value=KOUTP_sigRecircStSet_enum_ovrdflg
      link override Signal_Override/_ovrdval: Value=KOUTP_sigRecircStSet_enum_ovrdval
  VTHC_sigRecircSt_flg_Inproc : FVT_lib/outp/OverrideAndLimit  SystemSampleTime=-1  VariantActivationTime=update diagram  Latency=0  AutoFrameSizeCalculation=off
      link override Signal_Limit/_maxval: Value=KOUTP_sigRecircSt_flg_maxval
      link override Signal_Limit/_minval: Value=KOUTP_sigRecircSt_flg_minval
      link override Signal_Override/_ovrdflg: Value=KOUTP_sigRecircSt_flg_ovrdflg
      link override Signal_Override/_ovrdval: Value=KOUTP_sigRecircSt_flg_ovrdval
  VTHC_sigSetTempZon1St_C_Inproc : FVT_lib/outp/OverrideAndLimit  SystemSampleTime=-1  VariantActivationTime=update diagram  Latency=0  AutoFrameSizeCalculation=off
      link override Signal_Limit/_maxval: Value=KOUTP_sigSetTempZon1St_C_maxval
      link override Signal_Limit/_minval: Value=KOUTP_sigSetTempZon1St_C_minval
      link override Signal_Override/_ovrdflg: Value=KOUTP_sigSetTempZon1St_C_ovrdflg
      link override Signal_Override/_ovrdval: Value=KOUTP_sigSetTempZon1St_C_ovrdval
  VTHC_sigSetTempZon2StM_C_Inproc : FVT_lib/outp/OverrideAndLimit  SystemSampleTime=-1  VariantActivationTime=update diagram  Latency=0  AutoFrameSizeCalculation=off
      link override Signal_Limit/_maxval: Value=KOUTP_sigSetTempZon2StM_C_maxval
      link override Signal_Limit/_minval: Value=KOUTP_sigSetTempZon2StM_C_minval
      link override Signal_Override/_ovrdflg: Value=KOUTP_sigSetTempZon2StM_C_ovrdflg
      link override Signal_Override/_ovrdval: Value=KOUTP_sigSetTempZon2StM_C_ovrdval
  VTHC_sigSetTempZon2St_C_Inproc : FVT_lib/outp/OverrideAndLimit  SystemSampleTime=-1  VariantActivationTime=update diagram  Latency=0  AutoFrameSizeCalculation=off
      link override Signal_Limit/_maxval: Value=KOUTP_sigSetTempZon2St_C_maxval
      link override Signal_Limit/_minval: Value=KOUTP_sigSetTempZon2St_C_minval
      link override Signal_Override/_ovrdflg: Value=KOUTP_sigSetTempZon2St_C_ovrdflg
      link override Signal_Override/_ovrdval: Value=KOUTP_sigSetTempZon2St_C_ovrdval
  VTHC_sigWindDirZon1St_enum_Inproc : FVT_lib/outp/OverrideAndLimit  SystemSampleTime=-1  VariantActivationTime=update diagram  Latency=0  AutoFrameSizeCalculation=off
      link override Signal_Limit/_maxval: Value=KOUTP_sigWindDirZon1St_enum_maxval
      link override Signal_Limit/_minval: Value=KOUTP_sigWindDirZon1St_enum_minval
      link override Signal_Override/_ovrdflg: Value=KOUTP_sigWindDirZon1St_enum_ovrdflg
      link override Signal_Override/_ovrdval: Value=KOUTP_sigWindDirZon1St_enum_ovrdval
  VTPM_ALFin_flg_Inproc : FVT_lib/outp/OverrideAndLimit  SystemSampleTime=-1  VariantActivationTime=update diagram  Latency=0  AutoFrameSizeCalculation=off
      link override Signal_Limit/_maxval: Value=KOUTP_ALFin_flg_maxval
      link override Signal_Limit/_minval: Value=KOUTP_ALFin_flg_minval
      link override Signal_Override/_ovrdflg: Value=KOUTP_ALFin_flg_ovrdflg
      link override Signal_Override/_ovrdval: Value=KOUTP_ALFin_flg_ovrdval
  VTPM_AutoLTips_enum_Inproc : FVT_lib/outp/OverrideAndLimit  SystemSampleTime=-1  VariantActivationTime=update diagram  Latency=0  AutoFrameSizeCalculation=off
      link override Signal_Limit/_maxval: Value=KOUTP_AutoLTips_enum_maxval
      link override Signal_Limit/_minval: Value=KOUTP_AutoLTips_enum_minval
      link override Signal_Override/_ovrdflg: Value=KOUTP_AutoLTips_enum_ovrdflg
      link override Signal_Override/_ovrdval: Value=KOUTP_AutoLTips_enum_ovrdval
  VTPM_CWheelTips_enum_Inproc : FVT_lib/outp/OverrideAndLimit  SystemSampleTime=-1  VariantActivationTime=update diagram  Latency=0  AutoFrameSizeCalculation=off
      link override Signal_Limit/_maxval: Value=KOUTP_CWheelTips_enum_maxval
      link override Signal_Limit/_minval: Value=KOUTP_CWheelTips_enum_minval
      link override Signal_Override/_ovrdflg: Value=KOUTP_CWheelTips_enum_ovrdflg
      link override Signal_Override/_ovrdval: Value=KOUTP_CWheelTips_enum_ovrdval
  VTPM_ChkStorge_flg_Inproc : FVT_lib/outp/OverrideAndLimit  SystemSampleTime=-1  VariantActivationTime=update diagram  Latency=0  AutoFrameSizeCalculation=off
      link override Signal_Limit/_maxval: Value=KOUTP_ChkStorge_flg_maxval
      link override Signal_Limit/_minval: Value=KOUTP_ChkStorge_flg_minval
      link override Signal_Override/_ovrdflg: Value=KOUTP_ChkStorge_flg_ovrdflg
      link override Signal_Override/_ovrdval: Value=KOUTP_ChkStorge_flg_ovrdval
  VTPM_Chkfin_flg_Inproc : FVT_lib/outp/OverrideAndLimit  SystemSampleTime=-1  VariantActivationTime=update diagram  Latency=0  AutoFrameSizeCalculation=off
      link override Signal_Limit/_maxval: Value=KOUTP_Chkfin_flg_maxval
      link override Signal_Limit/_minval: Value=KOUTP_Chkfin_flg_minval
      link override Signal_Override/_ovrdflg: Value=KOUTP_Chkfin_flg_ovrdflg
      link override Signal_Override/_ovrdval: Value=KOUTP_Chkfin_flg_ovrdval
  VTPM_FAT_flg_Inproc : FVT_lib/outp/OverrideAndLimit  SystemSampleTime=-1  VariantActivationTime=update diagram  Latency=0  AutoFrameSizeCalculation=off
      link override Signal_Limit/_maxval: Value=KOUTP_FAT_flg_maxval
      link override Signal_Limit/_minval: Value=KOUTP_FAT_flg_minval
      link override Signal_Override/_ovrdflg: Value=KOUTP_FAT_flg_ovrdflg
      link override Signal_Override/_ovrdval: Value=KOUTP_FAT_flg_ovrdval
  VTPM_FlashIDvalid_enum_Inproc : FVT_lib/outp/OverrideAndLimit  SystemSampleTime=-1  VariantActivationTime=update diagram  Latency=0  AutoFrameSizeCalculation=off
      link override Signal_Limit/_maxval: Value=KOUTP_FlashIDvalid_enum_maxval
      link override Signal_Limit/_minval: Value=KOUTP_FlashIDvalid_enum_minval
      link override Signal_Override/_ovrdflg: Value=KOUTP_FlashIDvalid_enum_ovrdflg
      link override Signal_Override/_ovrdval: Value=KOUTP_FlashIDvalid_enum_ovrdval
  VTPM_FlashS1ID_raw_Inproc : FVT_lib/outp/OverrideAndLimit  SystemSampleTime=-1  VariantActivationTime=update diagram  Latency=0  AutoFrameSizeCalculation=off
      link override Signal_Limit/_maxval: Value=KOUTP_FlashS1ID_raw_maxval
      link override Signal_Limit/_minval: Value=KOUTP_FlashS1ID_raw_minval
      link override Signal_Override/_ovrdflg: Value=KOUTP_FlashS1ID_raw_ovrdflg
      link override Signal_Override/_ovrdval: Value=KOUTP_FlashS1ID_raw_ovrdval
  VTPM_FlashS2ID_raw_Inproc : FVT_lib/outp/OverrideAndLimit  SystemSampleTime=-1  VariantActivationTime=update diagram  Latency=0  AutoFrameSizeCalculation=off
      link override Signal_Limit/_maxval: Value=KOUTP_FlashS2ID_raw_maxval
      link override Signal_Limit/_minval: Value=KOUTP_FlashS2ID_raw_minval
      link override Signal_Override/_ovrdflg: Value=KOUTP_FlashS2ID_raw_ovrdflg
      link override Signal_Override/_ovrdval: Value=KOUTP_FlashS2ID_raw_ovrdval
  VTPM_FlashS3ID_raw_Inproc : FVT_lib/outp/OverrideAndLimit  SystemSampleTime=-1  VariantActivationTime=update diagram  Latency=0  AutoFrameSizeCalculation=off
      link override Signal_Limit/_maxval: Value=KOUTP_FlashS3ID_raw_maxval
      link override Signal_Limit/_minval: Value=KOUTP_FlashS3ID_raw_minval
      link override Signal_Override/_ovrdflg: Value=KOUTP_FlashS3ID_raw_ovrdflg
      link override Signal_Override/_ovrdval: Value=KOUTP_FlashS3ID_raw_ovrdval
  VTPM_FlashS4ID_raw_Inproc : FVT_lib/outp/OverrideAndLimit  SystemSampleTime=-1  VariantActivationTime=update diagram  Latency=0  AutoFrameSizeCalculation=off
      link override Signal_Limit/_maxval: Value=KOUTP_FlashS4ID_raw_maxval
      link override Signal_Limit/_minval: Value=KOUTP_FlashS4ID_raw_minval
      link override Signal_Override/_ovrdflg: Value=KOUTP_FlashS4ID_raw_ovrdflg
      link override Signal_Override/_ovrdval: Value=KOUTP_FlashS4ID_raw_ovrdval
  VTPM_Flashchkdatavalid_enum_Inproc : FVT_lib/outp/OverrideAndLimit  SystemSampleTime=-1  VariantActivationTime=update diagram  Latency=0  AutoFrameSizeCalculation=off
      link override Signal_Limit/_maxval: Value=KOUTP_Flashchkdatavalid_enum_maxval
      link override Signal_Limit/_minval: Value=KOUTP_Flashchkdatavalid_enum_minval
      link override Signal_Override/_ovrdflg: Value=KOUTP_Flashchkdatavalid_enum_ovrdflg
      link override Signal_Override/_ovrdval: Value=KOUTP_Flashchkdatavalid_enum_ovrdval
  VTPM_Flashdatavalid_enum_Inproc : FVT_lib/outp/OverrideAndLimit  SystemSampleTime=-1  VariantActivationTime=update diagram  Latency=0  AutoFrameSizeCalculation=off
      link override Signal_Limit/_maxval: Value=KOUTP_Flashdatavalid_enum_maxval
      link override Signal_Limit/_minval: Value=KOUTP_Flashdatavalid_enum_minval
      link override Signal_Override/_ovrdflg: Value=KOUTP_Flashdatavalid_enum_ovrdflg
      link override Signal_Override/_ovrdval: Value=KOUTP_Flashdatavalid_enum_ovrdval
  VTPM_ID1messageALTU_raw8_Inproc : FVT_lib/outp/OverrideAndLimit  SystemSampleTime=-1  VariantActivationTime=update diagram  Latency=0  AutoFrameSizeCalculation=off
      link override Signal_Limit/_maxval: Value=KOUTP_ID1messageALTU_raw8_maxval
      link override Signal_Limit/_minval: Value=KOUTP_ID1messageALTU_raw8_minval
      link override Signal_Override/_ovrdflg: Value=KOUTP_ID1messageALTU_raw8_ovrdflg
      link override Signal_Override/_ovrdval: Value=KOUTP_ID1messageALTU_raw8_ovrdval
  VTPM_ID2messageALTU_raw8_Inproc : FVT_lib/outp/OverrideAndLimit  SystemSampleTime=-1  VariantActivationTime=update diagram  Latency=0  AutoFrameSizeCalculation=off
      link override Signal_Limit/_maxval: Value=KOUTP_ID2messageALTU_raw8_maxval
      link override Signal_Limit/_minval: Value=KOUTP_ID2messageALTU_raw8_minval
      link override Signal_Override/_ovrdflg: Value=KOUTP_ID2messageALTU_raw8_ovrdflg
      link override Signal_Override/_ovrdval: Value=KOUTP_ID2messageALTU_raw8_ovrdval
  VTPM_ID3messageALTU_raw8_Inproc : FVT_lib/outp/OverrideAndLimit  SystemSampleTime=-1  VariantActivationTime=update diagram  Latency=0  AutoFrameSizeCalculation=off
      link override Signal_Limit/_maxval: Value=KOUTP_ID3messageALTU_raw8_maxval
      link override Signal_Limit/_minval: Value=KOUTP_ID3messageALTU_raw8_minval
      link override Signal_Override/_ovrdflg: Value=KOUTP_ID3messageALTU_raw8_ovrdflg
      link override Signal_Override/_ovrdval: Value=KOUTP_ID3messageALTU_raw8_ovrdval
  VTPM_ID4messageALTU_raw8_Inproc : FVT_lib/outp/OverrideAndLimit  SystemSampleTime=-1  VariantActivationTime=update diagram  Latency=0  AutoFrameSizeCalculation=off
      link override Signal_Limit/_maxval: Value=KOUTP_ID4messageALTU_raw8_maxval
      link override Signal_Limit/_minval: Value=KOUTP_ID4messageALTU_raw8_minval
      link override Signal_Override/_ovrdflg: Value=KOUTP_ID4messageALTU_raw8_ovrdflg
      link override Signal_Override/_ovrdval: Value=KOUTP_ID4messageALTU_raw8_ovrdval
  VTPM_IDin_raw32_Inproc : FVT_lib/outp/OverrideAndLimit  SystemSampleTime=-1  VariantActivationTime=update diagram  Latency=0  AutoFrameSizeCalculation=off
      link override Signal_Limit/_maxval: Value=KOUTP_IDin_raw32_maxval
      link override Signal_Limit/_minval: Value=KOUTP_IDin_raw32_minval
      link override Signal_Override/_ovrdflg: Value=KOUTP_IDin_raw32_ovrdflg
      link override Signal_Override/_ovrdval: Value=KOUTP_IDin_raw32_ovrdval
  VTPM_LFBatWarn_flg_Inproc : FVT_lib/outp/OverrideAndLimit  SystemSampleTime=-1  VariantActivationTime=update diagram  Latency=0  AutoFrameSizeCalculation=off
      link override Signal_Limit/_maxval: Value=KOUTP_LFBatWarn_flg_maxval
      link override Signal_Limit/_minval: Value=KOUTP_LFBatWarn_flg_minval
      link override Signal_Override/_ovrdflg: Value=KOUTP_LFBatWarn_flg_ovrdflg
      link override Signal_Override/_ovrdval: Value=KOUTP_LFBatWarn_flg_ovrdval
  VTPM_LFP20_raw8_Inproc : FVT_lib/outp/OverrideAndLimit  SystemSampleTime=-1  VariantActivationTime=update diagram  Latency=0  AutoFrameSizeCalculation=off
      link override Signal_Limit/_maxval: Value=KOUTP_LFP20_raw8_maxval
      link override Signal_Limit/_minval: Value=KOUTP_LFP20_raw8_minval
      link override Signal_Override/_ovrdflg: Value=KOUTP_LFP20_raw8_ovrdflg
      link override Signal_Override/_ovrdval: Value=KOUTP_LFP20_raw8_ovrdval
  VTPM_LFPindi_enum_Inproc : FVT_lib/outp/OverrideAndLimit  SystemSampleTime=-1  VariantActivationTime=update diagram  Latency=0  AutoFrameSizeCalculation=off
      link override Signal_Limit/_maxval: Value=KOUTP_LFPindi_enum_maxval
      link override Signal_Limit/_minval: Value=KOUTP_LFPindi_enum_minval
      link override Signal_Override/_ovrdflg: Value=KOUTP_LFPindi_enum_ovrdflg
      link override Signal_Override/_ovrdval: Value=KOUTP_LFPindi_enum_ovrdval
  VTPM_LFPressIndi_enum_Inproc : FVT_lib/outp/OverrideAndLimit  SystemSampleTime=-1  VariantActivationTime=update diagram  Latency=0  AutoFrameSizeCalculation=off
      link override Signal_Limit/_maxval: Value=KOUTP_LFPressIndi_enum_maxval
      link override Signal_Limit/_minval: Value=KOUTP_LFPressIndi_enum_minval
      link override Signal_Override/_ovrdflg: Value=KOUTP_LFPressIndi_enum_ovrdflg
      link override Signal_Override/_ovrdval: Value=KOUTP_LFPressIndi_enum_ovrdval
  VTPM_LFSensorFail_flg_Inproc : FVT_lib/outp/OverrideAndLimit  SystemSampleTime=-1  VariantActivationTime=update diagram  Latency=0  AutoFrameSizeCalculation=off
      link override Signal_Limit/_maxval: Value=KOUTP_LFSensorFail_flg_maxval
      link override Signal_Limit/_minval: Value=KOUTP_LFSensorFail_flg_minval
      link override Signal_Override/_ovrdflg: Value=KOUTP_LFSensorFail_flg_ovrdflg
      link override Signal_Override/_ovrdval: Value=KOUTP_LFSensorFail_flg_ovrdval
  VTPM_LFSensorMode_flg_Inproc : FVT_lib/outp/OverrideAndLimit  SystemSampleTime=-1  VariantActivationTime=update diagram  Latency=0  AutoFrameSizeCalculation=off
      link override Signal_Limit/_maxval: Value=KOUTP_LFSensorMode_flg_maxval
      link override Signal_Limit/_minval: Value=KOUTP_LFSensorMode_flg_minval
      link override Signal_Override/_ovrdflg: Value=KOUTP_LFSensorMode_flg_ovrdflg
      link override Signal_Override/_ovrdval: Value=KOUTP_LFSensorMode_flg_ovrdval
  VTPM_LFWheelDebug_flg_Inproc : FVT_lib/outp/OverrideAndLimit  SystemSampleTime=-1  VariantActivationTime=update diagram  Latency=0  AutoFrameSizeCalculation=off
      link override Signal_Limit/_maxval: Value=KOUTP_LFWheelDebug_flg_maxval
      link override Signal_Limit/_minval: Value=KOUTP_LFWheelDebug_flg_minval
      link override Signal_Override/_ovrdflg: Value=KOUTP_LFWheelDebug_flg_ovrdflg
      link override Signal_Override/_ovrdval: Value=KOUTP_LFWheelDebug_flg_ovrdval
  VTPM_LFWheelPSW_raw8_Inproc : FVT_lib/outp/OverrideAndLimit  SystemSampleTime=-1  VariantActivationTime=update diagram  Latency=0  AutoFrameSizeCalculation=off
      link override Signal_Limit/_maxval: Value=KOUTP_LFWheelPSW_raw8_maxval
      link override Signal_Limit/_minval: Value=KOUTP_LFWheelPSW_raw8_minval
      link override Signal_Override/_ovrdflg: Value=KOUTP_LFWheelPSW_raw8_ovrdflg
      link override Signal_Override/_ovrdval: Value=KOUTP_LFWheelPSW_raw8_ovrdval
  VTPM_LFWheelPress_raw8_Inproc : FVT_lib/outp/OverrideAndLimit  SystemSampleTime=-1  VariantActivationTime=update diagram  Latency=0  AutoFrameSizeCalculation=off
      link override Signal_Limit/_maxval: Value=KOUTP_LFWheelPress_raw8_maxval
      link override Signal_Limit/_minval: Value=KOUTP_LFWheelPress_raw8_minval
      link override Signal_Override/_ovrdflg: Value=KOUTP_LFWheelPress_raw8_ovrdflg
      link override Signal_Override/_ovrdval: Value=KOUTP_LFWheelPress_raw8_ovrdval
  VTPM_LFWheelTemp_C_Inproc : FVT_lib/outp/OverrideAndLimit  SystemSampleTime=-1  VariantActivationTime=update diagram  Latency=0  AutoFrameSizeCalculation=off
      link override Signal_Limit/_maxval: Value=KOUTP_LFWheelTemp_C_maxval
      link override Signal_Limit/_minval: Value=KOUTP_LFWheelTemp_C_minval
      link override Signal_Override/_ovrdflg: Value=KOUTP_LFWheelTemp_C_ovrdflg
      link override Signal_Override/_ovrdval: Value=KOUTP_LFWheelTemp_C_ovrdval
  VTPM_LFWheelTmpIndi_flg_Inproc : FVT_lib/outp/OverrideAndLimit  SystemSampleTime=-1  VariantActivationTime=update diagram  Latency=0  AutoFrameSizeCalculation=off
      link override Signal_Limit/_maxval: Value=KOUTP_LFWheelTmpIndi_flg_maxval
      link override Signal_Limit/_minval: Value=KOUTP_LFWheelTmpIndi_flg_minval
      link override Signal_Override/_ovrdflg: Value=KOUTP_LFWheelTmpIndi_flg_ovrdflg
      link override Signal_Override/_ovrdval: Value=KOUTP_LFWheelTmpIndi_flg_ovrdval
  VTPM_LProgress_enum_Inproc : FVT_lib/outp/OverrideAndLimit  SystemSampleTime=-1  VariantActivationTime=update diagram  Latency=0  AutoFrameSizeCalculation=off
      link override Signal_Limit/_maxval: Value=KOUTP_LProgress_enum_maxval
      link override Signal_Limit/_minval: Value=KOUTP_LProgress_enum_minval
      link override Signal_Override/_ovrdflg: Value=KOUTP_LProgress_enum_ovrdflg
      link override Signal_Override/_ovrdval: Value=KOUTP_LProgress_enum_ovrdval
  VTPM_LRBatWarn_flg_Inproc : FVT_lib/outp/OverrideAndLimit  SystemSampleTime=-1  VariantActivationTime=update diagram  Latency=0  AutoFrameSizeCalculation=off
      link override Signal_Limit/_maxval: Value=KOUTP_LRBatWarn_flg_maxval
      link override Signal_Limit/_minval: Value=KOUTP_LRBatWarn_flg_minval
      link override Signal_Override/_ovrdflg: Value=KOUTP_LRBatWarn_flg_ovrdflg
      link override Signal_Override/_ovrdval: Value=KOUTP_LRBatWarn_flg_ovrdval
  VTPM_LRP20_raw8_Inproc : FVT_lib/outp/OverrideAndLimit  SystemSampleTime=-1  VariantActivationTime=update diagram  Latency=0  AutoFrameSizeCalculation=off
      link override Signal_Limit/_maxval: Value=KOUTP_LRP20_raw8_maxval
      link override Signal_Limit/_minval: Value=KOUTP_LRP20_raw8_minval
      link override Signal_Override/_ovrdflg: Value=KOUTP_LRP20_raw8_ovrdflg
      link override Signal_Override/_ovrdval: Value=KOUTP_LRP20_raw8_ovrdval
  VTPM_LRPindi_enum_Inproc : FVT_lib/outp/OverrideAndLimit  SystemSampleTime=-1  VariantActivationTime=update diagram  Latency=0  AutoFrameSizeCalculation=off
      link override Signal_Limit/_maxval: Value=KOUTP_LRPindi_enum_maxval
      link override Signal_Limit/_minval: Value=KOUTP_LRPindi_enum_minval
      link override Signal_Override/_ovrdflg: Value=KOUTP_LRPindi_enum_ovrdflg
      link override Signal_Override/_ovrdval: Value=KOUTP_LRPindi_enum_ovrdval
  VTPM_LRPressIndi_enum_Inproc : FVT_lib/outp/OverrideAndLimit  SystemSampleTime=-1  VariantActivationTime=update diagram  Latency=0  AutoFrameSizeCalculation=off
      link override Signal_Limit/_maxval: Value=KOUTP_LRPressIndi_enum_maxval
      link override Signal_Limit/_minval: Value=KOUTP_LRPressIndi_enum_minval
      link override Signal_Override/_ovrdflg: Value=KOUTP_LRPressIndi_enum_ovrdflg
      link override Signal_Override/_ovrdval: Value=KOUTP_LRPressIndi_enum_ovrdval
  VTPM_LRSensorFail_flg_Inproc : FVT_lib/outp/OverrideAndLimit  SystemSampleTime=-1  VariantActivationTime=update diagram  Latency=0  AutoFrameSizeCalculation=off
      link override Signal_Limit/_maxval: Value=KOUTP_LRSensorFail_flg_maxval
      link override Signal_Limit/_minval: Value=KOUTP_LRSensorFail_flg_minval
      link override Signal_Override/_ovrdflg: Value=KOUTP_LRSensorFail_flg_ovrdflg
      link override Signal_Override/_ovrdval: Value=KOUTP_LRSensorFail_flg_ovrdval
  VTPM_LRSensorMode_flg_Inproc : FVT_lib/outp/OverrideAndLimit  SystemSampleTime=-1  VariantActivationTime=update diagram  Latency=0  AutoFrameSizeCalculation=off
      link override Signal_Limit/_maxval: Value=KOUTP_LRSensorMode_flg_maxval
      link override Signal_Limit/_minval: Value=KOUTP_LRSensorMode_flg_minval
      link override Signal_Override/_ovrdflg: Value=KOUTP_LRSensorMode_flg_ovrdflg
      link override Signal_Override/_ovrdval: Value=KOUTP_LRSensorMode_flg_ovrdval
  VTPM_LRWheelDebug_flg_Inproc : FVT_lib/outp/OverrideAndLimit  SystemSampleTime=-1  VariantActivationTime=update diagram  Latency=0  AutoFrameSizeCalculation=off
      link override Signal_Limit/_maxval: Value=KOUTP_LRWheelDebug_flg_maxval
      link override Signal_Limit/_minval: Value=KOUTP_LRWheelDebug_flg_minval
      link override Signal_Override/_ovrdflg: Value=KOUTP_LRWheelDebug_flg_ovrdflg
      link override Signal_Override/_ovrdval: Value=KOUTP_LRWheelDebug_flg_ovrdval
  VTPM_LRWheelPSW_raw8_Inproc : FVT_lib/outp/OverrideAndLimit  SystemSampleTime=-1  VariantActivationTime=update diagram  Latency=0  AutoFrameSizeCalculation=off
      link override Signal_Limit/_maxval: Value=KOUTP_LRWheelPSW_raw8_maxval
      link override Signal_Limit/_minval: Value=KOUTP_LRWheelPSW_raw8_minval
      link override Signal_Override/_ovrdflg: Value=KOUTP_LRWheelPSW_raw8_ovrdflg
      link override Signal_Override/_ovrdval: Value=KOUTP_LRWheelPSW_raw8_ovrdval
  VTPM_LRWheelPress_raw8_Inproc : FVT_lib/outp/OverrideAndLimit  SystemSampleTime=-1  VariantActivationTime=update diagram  Latency=0  AutoFrameSizeCalculation=off
      link override Signal_Limit/_maxval: Value=KOUTP_LRWheelPress_raw8_maxval
      link override Signal_Limit/_minval: Value=KOUTP_LRWheelPress_raw8_minval
      link override Signal_Override/_ovrdflg: Value=KOUTP_LRWheelPress_raw8_ovrdflg
      link override Signal_Override/_ovrdval: Value=KOUTP_LRWheelPress_raw8_ovrdval
  VTPM_LRWheelTemp_C_Inproc : FVT_lib/outp/OverrideAndLimit  SystemSampleTime=-1  VariantActivationTime=update diagram  Latency=0  AutoFrameSizeCalculation=off
      link override Signal_Limit/_maxval: Value=KOUTP_LRWheelTemp_C_maxval
      link override Signal_Limit/_minval: Value=KOUTP_LRWheelTemp_C_minval
      link override Signal_Override/_ovrdflg: Value=KOUTP_LRWheelTemp_C_ovrdflg
      link override Signal_Override/_ovrdval: Value=KOUTP_LRWheelTemp_C_ovrdval
  VTPM_LRWheelTmpIndi_flg_Inproc : FVT_lib/outp/OverrideAndLimit  SystemSampleTime=-1  VariantActivationTime=update diagram  Latency=0  AutoFrameSizeCalculation=off
      link override Signal_Limit/_maxval: Value=KOUTP_LRWheelTmpIndi_flg_maxval
      link override Signal_Limit/_minval: Value=KOUTP_LRWheelTmpIndi_flg_minval
      link override Signal_Override/_ovrdflg: Value=KOUTP_LRWheelTmpIndi_flg_ovrdflg
      link override Signal_Override/_ovrdval: Value=KOUTP_LRWheelTmpIndi_flg_ovrdval
  VTPM_ModelVersionChksum_raw_Inproc : FVT_lib/outp/OverrideAndLimit  SystemSampleTime=-1  VariantActivationTime=update diagram  Latency=0  AutoFrameSizeCalculation=off
      link override Signal_Limit/_maxval: Value=KOUTP_ModelVersionChksum_raw_maxval
      link override Signal_Limit/_minval: Value=KOUTP_ModelVersionChksum_raw_minval
      link override Signal_Override/_ovrdflg: Value=KOUTP_ModelVersionChksum_raw_ovrdflg
      link override Signal_Override/_ovrdval: Value=KOUTP_ModelVersionChksum_raw_ovrdval
  VTPM_ModelVersion_raw_Inproc : FVT_lib/outp/OverrideAndLimit  SystemSampleTime=-1  VariantActivationTime=update diagram  Latency=0  AutoFrameSizeCalculation=off
      link override Signal_Limit/_maxval: Value=KOUTP_ModelVersion_raw_maxval
      link override Signal_Limit/_minval: Value=KOUTP_ModelVersion_raw_minval
      link override Signal_Override/_ovrdflg: Value=KOUTP_ModelVersion_raw_ovrdflg
      link override Signal_Override/_ovrdval: Value=KOUTP_ModelVersion_raw_ovrdval
  VTPM_Prepresstempvalid_enum_Inproc : FVT_lib/outp/OverrideAndLimit  SystemSampleTime=-1  VariantActivationTime=update diagram  Latency=0  AutoFrameSizeCalculation=off
      link override Signal_Limit/_maxval: Value=KOUTP_Prepresstempvalid_enum_maxval
      link override Signal_Limit/_minval: Value=KOUTP_Prepresstempvalid_enum_minval
      link override Signal_Override/_ovrdflg: Value=KOUTP_Prepresstempvalid_enum_ovrdflg
      link override Signal_Override/_ovrdval: Value=KOUTP_Prepresstempvalid_enum_ovrdval
  VTPM_RFBatWarn_flg_Inproc : FVT_lib/outp/OverrideAndLimit  SystemSampleTime=-1  VariantActivationTime=update diagram  Latency=0  AutoFrameSizeCalculation=off
      link override Signal_Limit/_maxval: Value=KOUTP_RFBatWarn_flg_maxval
      link override Signal_Limit/_minval: Value=KOUTP_RFBatWarn_flg_minval
      link override Signal_Override/_ovrdflg: Value=KOUTP_RFBatWarn_flg_ovrdflg
      link override Signal_Override/_ovrdval: Value=KOUTP_RFBatWarn_flg_ovrdval
  VTPM_RFP20_raw8_Inproc : FVT_lib/outp/OverrideAndLimit  SystemSampleTime=-1  VariantActivationTime=update diagram  Latency=0  AutoFrameSizeCalculation=off
      link override Signal_Limit/_maxval: Value=KOUTP_RFP20_raw8_maxval
      link override Signal_Limit/_minval: Value=KOUTP_RFP20_raw8_minval
      link override Signal_Override/_ovrdflg: Value=KOUTP_RFP20_raw8_ovrdflg
      link override Signal_Override/_ovrdval: Value=KOUTP_RFP20_raw8_ovrdval
  VTPM_RFPind_enum_Inproc : FVT_lib/outp/OverrideAndLimit  SystemSampleTime=-1  VariantActivationTime=update diagram  Latency=0  AutoFrameSizeCalculation=off
      link override Signal_Limit/_maxval: Value=KOUTP_RFPind_enum_maxval
      link override Signal_Limit/_minval: Value=KOUTP_RFPind_enum_minval
      link override Signal_Override/_ovrdflg: Value=KOUTP_RFPind_enum_ovrdflg
      link override Signal_Override/_ovrdval: Value=KOUTP_RFPind_enum_ovrdval
  VTPM_RFPressIndi_enum_Inproc : FVT_lib/outp/OverrideAndLimit  SystemSampleTime=-1  VariantActivationTime=update diagram  Latency=0  AutoFrameSizeCalculation=off
      link override Signal_Limit/_maxval: Value=KOUTP_RFPressIndi_enum_maxval
      link override Signal_Limit/_minval: Value=KOUTP_RFPressIndi_enum_minval
      link override Signal_Override/_ovrdflg: Value=KOUTP_RFPressIndi_enum_ovrdflg
      link override Signal_Override/_ovrdval: Value=KOUTP_RFPressIndi_enum_ovrdval
  VTPM_RFSensorFail_flg_Inproc : FVT_lib/outp/OverrideAndLimit  SystemSampleTime=-1  VariantActivationTime=update diagram  Latency=0  AutoFrameSizeCalculation=off
      link override Signal_Limit/_maxval: Value=KOUTP_RFSensorFail_flg_maxval
      link override Signal_Limit/_minval: Value=KOUTP_RFSensorFail_flg_minval
      link override Signal_Override/_ovrdflg: Value=KOUTP_RFSensorFail_flg_ovrdflg
      link override Signal_Override/_ovrdval: Value=KOUTP_RFSensorFail_flg_ovrdval
  VTPM_RFSensorMode_flg_Inproc : FVT_lib/outp/OverrideAndLimit  SystemSampleTime=-1  VariantActivationTime=update diagram  Latency=0  AutoFrameSizeCalculation=off
      link override Signal_Limit/_maxval: Value=KOUTP_RFSensorMode_flg_maxval
      link override Signal_Limit/_minval: Value=KOUTP_RFSensorMode_flg_minval
      link override Signal_Override/_ovrdflg: Value=KOUTP_RFSensorMode_flg_ovrdflg
      link override Signal_Override/_ovrdval: Value=KOUTP_RFSensorMode_flg_ovrdval
  VTPM_RFWheelDebug_flg_Inproc : FVT_lib/outp/OverrideAndLimit  SystemSampleTime=-1  VariantActivationTime=update diagram  Latency=0  AutoFrameSizeCalculation=off
      link override Signal_Limit/_maxval: Value=KOUTP_RFWheelDebug_flg_maxval
      link override Signal_Limit/_minval: Value=KOUTP_RFWheelDebug_flg_minval
      link override Signal_Override/_ovrdflg: Value=KOUTP_RFWheelDebug_flg_ovrdflg
      link override Signal_Override/_ovrdval: Value=KOUTP_RFWheelDebug_flg_ovrdval
  VTPM_RFWheelPSW_raw8_Inproc : FVT_lib/outp/OverrideAndLimit  SystemSampleTime=-1  VariantActivationTime=update diagram  Latency=0  AutoFrameSizeCalculation=off
      link override Signal_Limit/_maxval: Value=KOUTP_RFWheelPSW_raw8_maxval
      link override Signal_Limit/_minval: Value=KOUTP_RFWheelPSW_raw8_minval
      link override Signal_Override/_ovrdflg: Value=KOUTP_RFWheelPSW_raw8_ovrdflg
      link override Signal_Override/_ovrdval: Value=KOUTP_RFWheelPSW_raw8_ovrdval
  VTPM_RFWheelPress_raw8_Inproc : FVT_lib/outp/OverrideAndLimit  SystemSampleTime=-1  VariantActivationTime=update diagram  Latency=0  AutoFrameSizeCalculation=off
      link override Signal_Limit/_maxval: Value=KOUTP_RFWheelPress_raw8_maxval
      link override Signal_Limit/_minval: Value=KOUTP_RFWheelPress_raw8_minval
      link override Signal_Override/_ovrdflg: Value=KOUTP_RFWheelPress_raw8_ovrdflg
      link override Signal_Override/_ovrdval: Value=KOUTP_RFWheelPress_raw8_ovrdval
  VTPM_RFWheelTemp_C_Inproc : FVT_lib/outp/OverrideAndLimit  SystemSampleTime=-1  VariantActivationTime=update diagram  Latency=0  AutoFrameSizeCalculation=off
      link override Signal_Limit/_maxval: Value=KOUTP_RFWheelTemp_C_maxval
      link override Signal_Limit/_minval: Value=KOUTP_RFWheelTemp_C_minval
      link override Signal_Override/_ovrdflg: Value=KOUTP_RFWheelTemp_C_ovrdflg
      link override Signal_Override/_ovrdval: Value=KOUTP_RFWheelTemp_C_ovrdval
  VTPM_RFWheelTmpIndi_flg_Inproc : FVT_lib/outp/OverrideAndLimit  SystemSampleTime=-1  VariantActivationTime=update diagram  Latency=0  AutoFrameSizeCalculation=off
      link override Signal_Limit/_maxval: Value=KOUTP_RFWheelTmpIndi_flg_maxval
      link override Signal_Limit/_minval: Value=KOUTP_RFWheelTmpIndi_flg_minval
      link override Signal_Override/_ovrdflg: Value=KOUTP_RFWheelTmpIndi_flg_ovrdflg
      link override Signal_Override/_ovrdval: Value=KOUTP_RFWheelTmpIndi_flg_ovrdval
  VTPM_RRBatWarn_flg_Inproc : FVT_lib/outp/OverrideAndLimit  SystemSampleTime=-1  VariantActivationTime=update diagram  Latency=0  AutoFrameSizeCalculation=off
      link override Signal_Limit/_maxval: Value=KOUTP_RRBatWarn_flg_maxval
      link override Signal_Limit/_minval: Value=KOUTP_RRBatWarn_flg_minval
      link override Signal_Override/_ovrdflg: Value=KOUTP_RRBatWarn_flg_ovrdflg
      link override Signal_Override/_ovrdval: Value=KOUTP_RRBatWarn_flg_ovrdval
  VTPM_RRP20_raw8_Inproc : FVT_lib/outp/OverrideAndLimit  SystemSampleTime=-1  VariantActivationTime=update diagram  Latency=0  AutoFrameSizeCalculation=off
      link override Signal_Limit/_maxval: Value=KOUTP_RRP20_raw8_maxval
      link override Signal_Limit/_minval: Value=KOUTP_RRP20_raw8_minval
      link override Signal_Override/_ovrdflg: Value=KOUTP_RRP20_raw8_ovrdflg
      link override Signal_Override/_ovrdval: Value=KOUTP_RRP20_raw8_ovrdval
  VTPM_RRPindi_enum_Inproc : FVT_lib/outp/OverrideAndLimit  SystemSampleTime=-1  VariantActivationTime=update diagram  Latency=0  AutoFrameSizeCalculation=off
      link override Signal_Limit/_maxval: Value=KOUTP_RRPindi_enum_maxval
      link override Signal_Limit/_minval: Value=KOUTP_RRPindi_enum_minval
      link override Signal_Override/_ovrdflg: Value=KOUTP_RRPindi_enum_ovrdflg
      link override Signal_Override/_ovrdval: Value=KOUTP_RRPindi_enum_ovrdval
  VTPM_RRPressIndi_enum_Inproc : FVT_lib/outp/OverrideAndLimit  SystemSampleTime=-1  VariantActivationTime=update diagram  Latency=0  AutoFrameSizeCalculation=off
      link override Signal_Limit/_maxval: Value=KOUTP_RRPressIndi_enum_maxval
      link override Signal_Limit/_minval: Value=KOUTP_RRPressIndi_enum_minval
      link override Signal_Override/_ovrdflg: Value=KOUTP_RRPressIndi_enum_ovrdflg
      link override Signal_Override/_ovrdval: Value=KOUTP_RRPressIndi_enum_ovrdval
  VTPM_RRSensorFail_flg_Inproc : FVT_lib/outp/OverrideAndLimit  SystemSampleTime=-1  VariantActivationTime=update diagram  Latency=0  AutoFrameSizeCalculation=off
      link override Signal_Limit/_maxval: Value=KOUTP_RRSensorFail_flg_maxval
      link override Signal_Limit/_minval: Value=KOUTP_RRSensorFail_flg_minval
      link override Signal_Override/_ovrdflg: Value=KOUTP_RRSensorFail_flg_ovrdflg
      link override Signal_Override/_ovrdval: Value=KOUTP_RRSensorFail_flg_ovrdval
  VTPM_RRSensorMode_flg_Inproc : FVT_lib/outp/OverrideAndLimit  SystemSampleTime=-1  VariantActivationTime=update diagram  Latency=0  AutoFrameSizeCalculation=off
      link override Signal_Limit/_maxval: Value=KOUTP_RRSensorMode_flg_maxval
      link override Signal_Limit/_minval: Value=KOUTP_RRSensorMode_flg_minval
      link override Signal_Override/_ovrdflg: Value=KOUTP_RRSensorMode_flg_ovrdflg
      link override Signal_Override/_ovrdval: Value=KOUTP_RRSensorMode_flg_ovrdval
  VTPM_RRWheelDebug_flg_Inproc : FVT_lib/outp/OverrideAndLimit  SystemSampleTime=-1  VariantActivationTime=update diagram  Latency=0  AutoFrameSizeCalculation=off
      link override Signal_Limit/_maxval: Value=KOUTP_RRWheelDebug_flg_maxval
      link override Signal_Limit/_minval: Value=KOUTP_RRWheelDebug_flg_minval
      link override Signal_Override/_ovrdflg: Value=KOUTP_RRWheelDebug_flg_ovrdflg
      link override Signal_Override/_ovrdval: Value=KOUTP_RRWheelDebug_flg_ovrdval
  VTPM_RRWheelPSW_raw8_Inproc : FVT_lib/outp/OverrideAndLimit  SystemSampleTime=-1  VariantActivationTime=update diagram  Latency=0  AutoFrameSizeCalculation=off
      link override Signal_Limit/_maxval: Value=KOUTP_RRWheelPSW_raw8_maxval
      link override Signal_Limit/_minval: Value=KOUTP_RRWheelPSW_raw8_minval
      link override Signal_Override/_ovrdflg: Value=KOUTP_RRWheelPSW_raw8_ovrdflg
      link override Signal_Override/_ovrdval: Value=KOUTP_RRWheelPSW_raw8_ovrdval
  VTPM_RRWheelPress_raw8_Inproc : FVT_lib/outp/OverrideAndLimit  SystemSampleTime=-1  VariantActivationTime=update diagram  Latency=0  AutoFrameSizeCalculation=off
      link override Signal_Limit/_maxval: Value=KOUTP_RRWheelPress_raw8_maxval
      link override Signal_Limit/_minval: Value=KOUTP_RRWheelPress_raw8_minval
      link override Signal_Override/_ovrdflg: Value=KOUTP_RRWheelPress_raw8_ovrdflg
      link override Signal_Override/_ovrdval: Value=KOUTP_RRWheelPress_raw8_ovrdval
  VTPM_RRWheelTemp_C_Inproc : FVT_lib/outp/OverrideAndLimit  SystemSampleTime=-1  VariantActivationTime=update diagram  Latency=0  AutoFrameSizeCalculation=off
      link override Signal_Limit/_maxval: Value=KOUTP_RRWheelTemp_C_maxval
      link override Signal_Limit/_minval: Value=KOUTP_RRWheelTemp_C_minval
      link override Signal_Override/_ovrdflg: Value=KOUTP_RRWheelTemp_C_ovrdflg
      link override Signal_Override/_ovrdval: Value=KOUTP_RRWheelTemp_C_ovrdval
  VTPM_RRWheelTmpIndi_flg_Inproc : FVT_lib/outp/OverrideAndLimit  SystemSampleTime=-1  VariantActivationTime=update diagram  Latency=0  AutoFrameSizeCalculation=off
      link override Signal_Limit/_maxval: Value=KOUTP_RRWheelTmpIndi_flg_maxval
      link override Signal_Limit/_minval: Value=KOUTP_RRWheelTmpIndi_flg_minval
      link override Signal_Override/_ovrdflg: Value=KOUTP_RRWheelTmpIndi_flg_ovrdflg
      link override Signal_Override/_ovrdval: Value=KOUTP_RRWheelTmpIndi_flg_ovrdval
  VTPM_S1ID_raw32_Inproc : FVT_lib/outp/OverrideAndLimit  SystemSampleTime=-1  VariantActivationTime=update diagram  Latency=0  AutoFrameSizeCalculation=off
      link override Signal_Limit/_maxval: Value=KOUTP_S1ID_raw32_maxval
      link override Signal_Limit/_minval: Value=KOUTP_S1ID_raw32_minval
      link override Signal_Override/_ovrdflg: Value=KOUTP_S1ID_raw32_ovrdflg
      link override Signal_Override/_ovrdval: Value=KOUTP_S1ID_raw32_ovrdval
  VTPM_S1L_enum_Inproc : FVT_lib/outp/OverrideAndLimit  SystemSampleTime=-1  VariantActivationTime=update diagram  Latency=0  AutoFrameSizeCalculation=off
      link override Signal_Limit/_maxval: Value=KOUTP_S1L_enum_maxval
      link override Signal_Limit/_minval: Value=KOUTP_S1L_enum_minval
      link override Signal_Override/_ovrdflg: Value=KOUTP_S1L_enum_ovrdflg
      link override Signal_Override/_ovrdval: Value=KOUTP_S1L_enum_ovrdval
  VTPM_S1WheelDebugALTU_pct_Inproc : FVT_lib/outp/OverrideAndLimit  SystemSampleTime=-1  VariantActivationTime=update diagram  Latency=0  AutoFrameSizeCalculation=off
      link override Signal_Limit/_maxval: Value=KOUTP_S1WheelDebugALTU_pct_maxval
      link override Signal_Limit/_minval: Value=KOUTP_S1WheelDebugALTU_pct_minval
      link override Signal_Override/_ovrdflg: Value=KOUTP_S1WheelDebugALTU_pct_ovrdflg
      link override Signal_Override/_ovrdval: Value=KOUTP_S1WheelDebugALTU_pct_ovrdval
  VTPM_S2ID_raw32_Inproc : FVT_lib/outp/OverrideAndLimit  SystemSampleTime=-1  VariantActivationTime=update diagram  Latency=0  AutoFrameSizeCalculation=off
      link override Signal_Limit/_maxval: Value=KOUTP_S2ID_raw32_maxval
      link override Signal_Limit/_minval: Value=KOUTP_S2ID_raw32_minval
      link override Signal_Override/_ovrdflg: Value=KOUTP_S2ID_raw32_ovrdflg
      link override Signal_Override/_ovrdval: Value=KOUTP_S2ID_raw32_ovrdval
  VTPM_S2L_enum_Inproc : FVT_lib/outp/OverrideAndLimit  SystemSampleTime=-1  VariantActivationTime=update diagram  Latency=0  AutoFrameSizeCalculation=off
      link override Signal_Limit/_maxval: Value=KOUTP_S2L_enum_maxval
      link override Signal_Limit/_minval: Value=KOUTP_S2L_enum_minval
      link override Signal_Override/_ovrdflg: Value=KOUTP_S2L_enum_ovrdflg
      link override Signal_Override/_ovrdval: Value=KOUTP_S2L_enum_ovrdval
  VTPM_S2WheelDebugALTU_pct_Inproc : FVT_lib/outp/OverrideAndLimit  SystemSampleTime=-1  VariantActivationTime=update diagram  Latency=0  AutoFrameSizeCalculation=off
      link override Signal_Limit/_maxval: Value=KOUTP_S2WheelDebugALTU_pct_maxval
      link override Signal_Limit/_minval: Value=KOUTP_S2WheelDebugALTU_pct_minval
      link override Signal_Override/_ovrdflg: Value=KOUTP_S2WheelDebugALTU_pct_ovrdflg
      link override Signal_Override/_ovrdval: Value=KOUTP_S2WheelDebugALTU_pct_ovrdval
  VTPM_S3ID_raw32_Inproc : FVT_lib/outp/OverrideAndLimit  SystemSampleTime=-1  VariantActivationTime=update diagram  Latency=0  AutoFrameSizeCalculation=off
      link override Signal_Limit/_maxval: Value=KOUTP_S3ID_raw32_maxval
      link override Signal_Limit/_minval: Value=KOUTP_S3ID_raw32_minval
      link override Signal_Override/_ovrdflg: Value=KOUTP_S3ID_raw32_ovrdflg
      link override Signal_Override/_ovrdval: Value=KOUTP_S3ID_raw32_ovrdval
  VTPM_S3L_enum_Inproc : FVT_lib/outp/OverrideAndLimit  SystemSampleTime=-1  VariantActivationTime=update diagram  Latency=0  AutoFrameSizeCalculation=off
      link override Signal_Limit/_maxval: Value=KOUTP_S3L_enum_maxval
      link override Signal_Limit/_minval: Value=KOUTP_S3L_enum_minval
      link override Signal_Override/_ovrdflg: Value=KOUTP_S3L_enum_ovrdflg
      link override Signal_Override/_ovrdval: Value=KOUTP_S3L_enum_ovrdval
  VTPM_S3WheelDebugALTU_pct_Inproc : FVT_lib/outp/OverrideAndLimit  SystemSampleTime=-1  VariantActivationTime=update diagram  Latency=0  AutoFrameSizeCalculation=off
      link override Signal_Limit/_maxval: Value=KOUTP_S3WheelDebugALTU_pct_maxval
      link override Signal_Limit/_minval: Value=KOUTP_S3WheelDebugALTU_pct_minval
      link override Signal_Override/_ovrdflg: Value=KOUTP_S3WheelDebugALTU_pct_ovrdflg
      link override Signal_Override/_ovrdval: Value=KOUTP_S3WheelDebugALTU_pct_ovrdval
  VTPM_S4ID_raw32_Inproc : FVT_lib/outp/OverrideAndLimit  SystemSampleTime=-1  VariantActivationTime=update diagram  Latency=0  AutoFrameSizeCalculation=off
      link override Signal_Limit/_maxval: Value=KOUTP_S4ID_raw32_maxval
      link override Signal_Limit/_minval: Value=KOUTP_S4ID_raw32_minval
      link override Signal_Override/_ovrdflg: Value=KOUTP_S4ID_raw32_ovrdflg
      link override Signal_Override/_ovrdval: Value=KOUTP_S4ID_raw32_ovrdval
  VTPM_S4L_enum_Inproc : FVT_lib/outp/OverrideAndLimit  SystemSampleTime=-1  VariantActivationTime=update diagram  Latency=0  AutoFrameSizeCalculation=off
      link override Signal_Limit/_maxval: Value=KOUTP_S4L_enum_maxval
      link override Signal_Limit/_minval: Value=KOUTP_S4L_enum_minval
      link override Signal_Override/_ovrdflg: Value=KOUTP_S4L_enum_ovrdflg
      link override Signal_Override/_ovrdval: Value=KOUTP_S4L_enum_ovrdval
  VTPM_S4WheelDebugALTU_pct_Inproc : FVT_lib/outp/OverrideAndLimit  SystemSampleTime=-1  VariantActivationTime=update diagram  Latency=0  AutoFrameSizeCalculation=off
      link override Signal_Limit/_maxval: Value=KOUTP_S4WheelDebugALTU_pct_maxval
      link override Signal_Limit/_minval: Value=KOUTP_S4WheelDebugALTU_pct_minval
      link override Signal_Override/_ovrdflg: Value=KOUTP_S4WheelDebugALTU_pct_ovrdflg
      link override Signal_Override/_ovrdval: Value=KOUTP_S4WheelDebugALTU_pct_ovrdval
  VTPM_SetIDLoc_flg_Inproc : FVT_lib/outp/OverrideAndLimit  SystemSampleTime=-1  VariantActivationTime=update diagram  Latency=0  AutoFrameSizeCalculation=off
      link override Signal_Limit/_maxval: Value=KOUTP_SetIDLoc_flg_maxval
      link override Signal_Limit/_minval: Value=KOUTP_SetIDLoc_flg_minval
      link override Signal_Override/_ovrdflg: Value=KOUTP_SetIDLoc_flg_ovrdflg
      link override Signal_Override/_ovrdval: Value=KOUTP_SetIDLoc_flg_ovrdval
  VTPM_TPMSCaliButtAllow_flg_Inproc : FVT_lib/outp/OverrideAndLimit  SystemSampleTime=-1  VariantActivationTime=update diagram  Latency=0  AutoFrameSizeCalculation=off
      link override Signal_Limit/_maxval: Value=KOUTP_TPMSCaliButtAllow_flg_maxval
      link override Signal_Limit/_minval: Value=KOUTP_TPMSCaliButtAllow_flg_minval
      link override Signal_Override/_ovrdflg: Value=KOUTP_TPMSCaliButtAllow_flg_ovrdflg
      link override Signal_Override/_ovrdval: Value=KOUTP_TPMSCaliButtAllow_flg_ovrdval
  VTPM_TPMSResButtAllow_flg_Inproc : FVT_lib/outp/OverrideAndLimit  SystemSampleTime=-1  VariantActivationTime=update diagram  Latency=0  AutoFrameSizeCalculation=off
      link override Signal_Limit/_maxval: Value=KOUTP_TPMSResButtAllow_flg_maxval
      link override Signal_Limit/_minval: Value=KOUTP_TPMSResButtAllow_flg_minval
      link override Signal_Override/_ovrdflg: Value=KOUTP_TPMSResButtAllow_flg_ovrdflg
      link override Signal_Override/_ovrdval: Value=KOUTP_TPMSResButtAllow_flg_ovrdval
  VTPM_TPMSResButt_flg_Inproc : FVT_lib/outp/OverrideAndLimit  SystemSampleTime=-1  VariantActivationTime=update diagram  Latency=0  AutoFrameSizeCalculation=off
      link override Signal_Limit/_maxval: Value=KOUTP_TPMSResButt_flg_maxval
      link override Signal_Limit/_minval: Value=KOUTP_TPMSResButt_flg_minval
      link override Signal_Override/_ovrdflg: Value=KOUTP_TPMSResButt_flg_ovrdflg
      link override Signal_Override/_ovrdval: Value=KOUTP_TPMSResButt_flg_ovrdval
  VTPM_TPMSSensorIDRegStart_flg_Inproc : FVT_lib/outp/OverrideAndLimit  SystemSampleTime=-1  VariantActivationTime=update diagram  Latency=0  AutoFrameSizeCalculation=off
      link override Signal_Limit/_maxval: Value=KOUTP_TPMSSensorIDRegStart_flg_maxval
      link override Signal_Limit/_minval: Value=KOUTP_TPMSSensorIDRegStart_flg_minval
      link override Signal_Override/_ovrdflg: Value=KOUTP_TPMSSensorIDRegStart_flg_ovrdflg
      link override Signal_Override/_ovrdval: Value=KOUTP_TPMSSensorIDRegStart_flg_ovrdval
  VTPM_TPMSStorge_flg_Inproc : FVT_lib/outp/OverrideAndLimit  SystemSampleTime=-1  VariantActivationTime=update diagram  Latency=0  AutoFrameSizeCalculation=off
      link override Signal_Limit/_maxval: Value=KOUTP_TPMSStorge_flg_maxval
      link override Signal_Limit/_minval: Value=KOUTP_TPMSStorge_flg_minval
      link override Signal_Override/_ovrdflg: Value=KOUTP_TPMSStorge_flg_ovrdflg
      link override Signal_Override/_ovrdval: Value=KOUTP_TPMSStorge_flg_ovrdval
  VTPM_TPMSTLCmd_flg_Inproc : FVT_lib/outp/OverrideAndLimit  SystemSampleTime=-1  VariantActivationTime=update diagram  Latency=0  AutoFrameSizeCalculation=off
      link override Signal_Limit/_maxval: Value=KOUTP_TPMSTLCmd_flg_maxval
      link override Signal_Limit/_minval: Value=KOUTP_TPMSTLCmd_flg_minval
      link override Signal_Override/_ovrdflg: Value=KOUTP_TPMSTLCmd_flg_ovrdflg
      link override Signal_Override/_ovrdval: Value=KOUTP_TPMSTLCmd_flg_ovrdval
  VTPM_TPMSWarnIndi_enum_Inproc : FVT_lib/outp/OverrideAndLimit  SystemSampleTime=-1  VariantActivationTime=update diagram  Latency=0  AutoFrameSizeCalculation=off
      link override Signal_Limit/_maxval: Value=KOUTP_TPMSWarnIndi_enum_maxval
      link override Signal_Limit/_minval: Value=KOUTP_TPMSWarnIndi_enum_minval
      link override Signal_Override/_ovrdflg: Value=KOUTP_TPMSWarnIndi_enum_ovrdflg
      link override Signal_Override/_ovrdval: Value=KOUTP_TPMSWarnIndi_enum_ovrdval
  VTPM_WriteChkLFID_raw_Inproc : FVT_lib/outp/OverrideAndLimit  SystemSampleTime=-1  VariantActivationTime=update diagram  Latency=0  AutoFrameSizeCalculation=off
      link override Signal_Limit/_maxval: Value=KOUTP_WriteChkLFID_raw_maxval
      link override Signal_Limit/_minval: Value=KOUTP_WriteChkLFID_raw_minval
      link override Signal_Override/_ovrdflg: Value=KOUTP_WriteChkLFID_raw_ovrdflg
      link override Signal_Override/_ovrdval: Value=KOUTP_WriteChkLFID_raw_ovrdval
  VTPM_WriteChkLRID_raw_Inproc : FVT_lib/outp/OverrideAndLimit  SystemSampleTime=-1  VariantActivationTime=update diagram  Latency=0  AutoFrameSizeCalculation=off
      link override Signal_Limit/_maxval: Value=KOUTP_WriteChkLRID_raw_maxval
      link override Signal_Limit/_minval: Value=KOUTP_WriteChkLRID_raw_minval
      link override Signal_Override/_ovrdflg: Value=KOUTP_WriteChkLRID_raw_ovrdflg
      link override Signal_Override/_ovrdval: Value=KOUTP_WriteChkLRID_raw_ovrdval
  VTPM_WriteChkRFID_raw_Inproc : FVT_lib/outp/OverrideAndLimit  SystemSampleTime=-1  VariantActivationTime=update diagram  Latency=0  AutoFrameSizeCalculation=off
      link override Signal_Limit/_maxval: Value=KOUTP_WriteChkRFID_raw_maxval
      link override Signal_Limit/_minval: Value=KOUTP_WriteChkRFID_raw_minval
      link override Signal_Override/_ovrdflg: Value=KOUTP_WriteChkRFID_raw_ovrdflg
      link override Signal_Override/_ovrdval: Value=KOUTP_WriteChkRFID_raw_ovrdval
  VTPM_WriteChkRRID_raw_Inproc : FVT_lib/outp/OverrideAndLimit  SystemSampleTime=-1  VariantActivationTime=update diagram  Latency=0  AutoFrameSizeCalculation=off
      link override Signal_Limit/_maxval: Value=KOUTP_WriteChkRRID_raw_maxval
      link override Signal_Limit/_minval: Value=KOUTP_WriteChkRRID_raw_minval
      link override Signal_Override/_ovrdflg: Value=KOUTP_WriteChkRRID_raw_ovrdflg
      link override Signal_Override/_ovrdval: Value=KOUTP_WriteChkRRID_raw_ovrdval
  VTPM_WriteChkfinLFID_raw_Inproc : FVT_lib/outp/OverrideAndLimit  SystemSampleTime=-1  VariantActivationTime=update diagram  Latency=0  AutoFrameSizeCalculation=off
      link override Signal_Limit/_maxval: Value=KOUTP_WriteChkfinLFID_raw_maxval
      link override Signal_Limit/_minval: Value=KOUTP_WriteChkfinLFID_raw_minval
      link override Signal_Override/_ovrdflg: Value=KOUTP_WriteChkfinLFID_raw_ovrdflg
      link override Signal_Override/_ovrdval: Value=KOUTP_WriteChkfinLFID_raw_ovrdval
  VTPM_WriteChkfinLRID_raw_Inproc : FVT_lib/outp/OverrideAndLimit  SystemSampleTime=-1  VariantActivationTime=update diagram  Latency=0  AutoFrameSizeCalculation=off
      link override Signal_Limit/_maxval: Value=KOUTP_WriteChkfinLRID_raw_maxval
      link override Signal_Limit/_minval: Value=KOUTP_WriteChkfinLRID_raw_minval
      link override Signal_Override/_ovrdflg: Value=KOUTP_WriteChkfinLRID_raw_ovrdflg
      link override Signal_Override/_ovrdval: Value=KOUTP_WriteChkfinLRID_raw_ovrdval
  VTPM_WriteChkfinRFID_raw_Inproc : FVT_lib/outp/OverrideAndLimit  SystemSampleTime=-1  VariantActivationTime=update diagram  Latency=0  AutoFrameSizeCalculation=off
      link override Signal_Limit/_maxval: Value=KOUTP_WriteChkfinRFID_raw_maxval
      link override Signal_Limit/_minval: Value=KOUTP_WriteChkfinRFID_raw_minval
      link override Signal_Override/_ovrdflg: Value=KOUTP_WriteChkfinRFID_raw_ovrdflg
      link override Signal_Override/_ovrdval: Value=KOUTP_WriteChkfinRFID_raw_ovrdval
  VTPM_WriteChkfinRRID_raw_Inproc : FVT_lib/outp/OverrideAndLimit  SystemSampleTime=-1  VariantActivationTime=update diagram  Latency=0  AutoFrameSizeCalculation=off
      link override Signal_Limit/_maxval: Value=KOUTP_WriteChkfinRRID_raw_maxval
      link override Signal_Limit/_minval: Value=KOUTP_WriteChkfinRRID_raw_minval
      link override Signal_Override/_ovrdflg: Value=KOUTP_WriteChkfinRRID_raw_ovrdflg
      link override Signal_Override/_ovrdval: Value=KOUTP_WriteChkfinRRID_raw_ovrdval
  VTPM_WritingCnt_enum_Inproc : FVT_lib/outp/OverrideAndLimit  SystemSampleTime=-1  VariantActivationTime=update diagram  Latency=0  AutoFrameSizeCalculation=off
      link override Signal_Limit/_maxval: Value=KOUTP_WritingCnt_enum_maxval
      link override Signal_Limit/_minval: Value=KOUTP_WritingCnt_enum_minval
      link override Signal_Override/_ovrdflg: Value=KOUTP_WritingCnt_enum_ovrdflg
      link override Signal_Override/_ovrdval: Value=KOUTP_WritingCnt_enum_ovrdval
  VTPM_unlearnSfailvalid_enum_Inproc : FVT_lib/outp/OverrideAndLimit  SystemSampleTime=-1  VariantActivationTime=update diagram  Latency=0  AutoFrameSizeCalculation=off
      link override Signal_Limit/_maxval: Value=KOUTP_unlearnSfailvalid_enum_maxval
      link override Signal_Limit/_minval: Value=KOUTP_unlearnSfailvalid_enum_minval
      link override Signal_Override/_ovrdflg: Value=KOUTP_unlearnSfailvalid_enum_ovrdflg
      link override Signal_Override/_ovrdval: Value=KOUTP_unlearnSfailvalid_enum_ovrdval
  VTPM_unlearnSfali_flg_Inproc : FVT_lib/outp/OverrideAndLimit  SystemSampleTime=-1  VariantActivationTime=update diagram  Latency=0  AutoFrameSizeCalculation=off
      link override Signal_Limit/_maxval: Value=KOUTP_unlearnSfali_flg_maxval
      link override Signal_Limit/_minval: Value=KOUTP_unlearnSfali_flg_minval
      link override Signal_Override/_ovrdflg: Value=KOUTP_unlearnSfali_flg_ovrdflg
      link override Signal_Override/_ovrdval: Value=KOUTP_unlearnSfali_flg_ovrdval
  VTQD_ActParkRequest_flg_Inproc : FVT_lib/outp/OverrideAndLimit  SystemSampleTime=-1  VariantActivationTime=update diagram  Latency=0  AutoFrameSizeCalculation=off
      link override Signal_Limit/_maxval: Value=KOUTP_ActParkRequest_flg_maxval
      link override Signal_Limit/_minval: Value=KOUTP_ActParkRequest_flg_minval
      link override Signal_Override/_ovrdflg: Value=KOUTP_ActParkRequest_flg_ovrdflg
      link override Signal_Override/_ovrdval: Value=KOUTP_ActParkRequest_flg_ovrdval
  VTQD_BOSEnable_flg_Inproc : FVT_lib/outp/OverrideAndLimit  SystemSampleTime=-1  VariantActivationTime=update diagram  Latency=0  AutoFrameSizeCalculation=off
      link override Signal_Limit/_maxval: Value=KOUTP_BOSEnable_flg_maxval
      link override Signal_Limit/_minval: Value=KOUTP_BOSEnable_flg_minval
      link override Signal_Override/_ovrdflg: Value=KOUTP_BOSEnable_flg_ovrdflg
      link override Signal_Override/_ovrdval: Value=KOUTP_BOSEnable_flg_ovrdval
  VTQD_CreepON_flg_Inproc : FVT_lib/outp/OverrideAndLimit  SystemSampleTime=-1  VariantActivationTime=update diagram  Latency=0  AutoFrameSizeCalculation=off
      link override Signal_Limit/_maxval: Value=KOUTP_CreepON_flg_maxval
      link override Signal_Limit/_minval: Value=KOUTP_CreepON_flg_minval
      link override Signal_Override/_ovrdflg: Value=KOUTP_CreepON_flg_ovrdflg
      link override Signal_Override/_ovrdval: Value=KOUTP_CreepON_flg_ovrdval
  VTQD_DriveProtEn_flg_Inproc : FVT_lib/outp/OverrideAndLimit  SystemSampleTime=-1  VariantActivationTime=update diagram  Latency=0  AutoFrameSizeCalculation=off
      link override Signal_Limit/_maxval: Value=KOUTP_DriveProtEn_flg_maxval
      link override Signal_Limit/_minval: Value=KOUTP_DriveProtEn_flg_minval
      link override Signal_Override/_ovrdflg: Value=KOUTP_DriveProtEn_flg_ovrdflg
      link override Signal_Override/_ovrdval: Value=KOUTP_DriveProtEn_flg_ovrdval
  VTQD_DriverWhlTqDemFr_Nm_Inproc : FVT_lib/outp/OverrideAndLimit  SystemSampleTime=-1  VariantActivationTime=update diagram  Latency=0  AutoFrameSizeCalculation=off
      link override Signal_Limit/_maxval: Value=KOUTP_DriverWhlTqDemFr_Nm_maxval
      link override Signal_Limit/_minval: Value=KOUTP_DriverWhlTqDemFr_Nm_minval
      link override Signal_Override/_ovrdflg: Value=KOUTP_DriverWhlTqDemFr_Nm_ovrdflg
      link override Signal_Override/_ovrdval: Value=KOUTP_DriverWhlTqDemFr_Nm_ovrdval
  VTQD_DriverWhlTqDemRr_Nm_Inproc : FVT_lib/outp/OverrideAndLimit  SystemSampleTime=-1  VariantActivationTime=update diagram  Latency=0  AutoFrameSizeCalculation=off
      link override Signal_Limit/_maxval: Value=KOUTP_DriverWhlTqDemRr_Nm_maxval
      link override Signal_Limit/_minval: Value=KOUTP_DriverWhlTqDemRr_Nm_minval
      link override Signal_Override/_ovrdflg: Value=KOUTP_DriverWhlTqDemRr_Nm_ovrdflg
      link override Signal_Override/_ovrdval: Value=KOUTP_DriverWhlTqDemRr_Nm_ovrdval
  VTQD_EVDriveMode_enum_Inproc : FVT_lib/outp/OverrideAndLimit  SystemSampleTime=-1  VariantActivationTime=update diagram  Latency=0  AutoFrameSizeCalculation=off
      link override Signal_Limit/_maxval: Value=KOUTP_EVDriveMode_enum_maxval
      link override Signal_Limit/_minval: Value=KOUTP_EVDriveMode_enum_minval
      link override Signal_Override/_ovrdflg: Value=KOUTP_EVDriveMode_enum_ovrdflg
      link override Signal_Override/_ovrdval: Value=KOUTP_EVDriveMode_enum_ovrdval
  VTQD_EquivAccPedalSWSta_flg_Inproc : FVT_lib/outp/OverrideAndLimit  SystemSampleTime=-1  VariantActivationTime=update diagram  Latency=0  AutoFrameSizeCalculation=off
      link override Signal_Limit/_maxval: Value=KOUTP_EquivAccPedalSWSta_flg_maxval
      link override Signal_Limit/_minval: Value=KOUTP_EquivAccPedalSWSta_flg_minval
      link override Signal_Override/_ovrdflg: Value=KOUTP_EquivAccPedalSWSta_flg_ovrdflg
      link override Signal_Override/_ovrdval: Value=KOUTP_EquivAccPedalSWSta_flg_ovrdval
  VTQD_FDCVCURegenMode_enum_Inproc : FVT_lib/outp/OverrideAndLimit  SystemSampleTime=-1  VariantActivationTime=update diagram  Latency=0  AutoFrameSizeCalculation=off
      link override Signal_Limit/_maxval: Value=KOUTP_FDCVCURegenMode_enum_maxval
      link override Signal_Limit/_minval: Value=KOUTP_FDCVCURegenMode_enum_minval
      link override Signal_Override/_ovrdflg: Value=KOUTP_FDCVCURegenMode_enum_ovrdflg
      link override Signal_Override/_ovrdval: Value=KOUTP_FDCVCURegenMode_enum_ovrdval
  VTQD_ForceP_flg_Inproc : FVT_lib/outp/OverrideAndLimit  SystemSampleTime=-1  VariantActivationTime=update diagram  Latency=0  AutoFrameSizeCalculation=off
      link override Signal_Limit/_maxval: Value=KOUTP_ForceP_flg_maxval
      link override Signal_Limit/_minval: Value=KOUTP_ForceP_flg_minval
      link override Signal_Override/_ovrdflg: Value=KOUTP_ForceP_flg_ovrdflg
      link override Signal_Override/_ovrdval: Value=KOUTP_ForceP_flg_ovrdval
  VTQD_FrActvDmpDisabReq_flg_Inproc : FVT_lib/outp/OverrideAndLimit  SystemSampleTime=-1  VariantActivationTime=update diagram  Latency=0  AutoFrameSizeCalculation=off
      link override Signal_Limit/_maxval: Value=KOUTP_FrActvDmpDisabReq_flg_maxval
      link override Signal_Limit/_minval: Value=KOUTP_FrActvDmpDisabReq_flg_minval
      link override Signal_Override/_ovrdflg: Value=KOUTP_FrActvDmpDisabReq_flg_ovrdflg
      link override Signal_Override/_ovrdval: Value=KOUTP_FrActvDmpDisabReq_flg_ovrdval
  VTQD_FrEDUActTq_Nm_Inproc : FVT_lib/outp/OverrideAndLimit  SystemSampleTime=-1  VariantActivationTime=update diagram  Latency=0  AutoFrameSizeCalculation=off
      link override Signal_Limit/_maxval: Value=KOUTP_FrEDUActTq_Nm_maxval
      link override Signal_Limit/_minval: Value=KOUTP_FrEDUActTq_Nm_minval
      link override Signal_Override/_ovrdflg: Value=KOUTP_FrEDUActTq_Nm_ovrdflg
      link override Signal_Override/_ovrdval: Value=KOUTP_FrEDUActTq_Nm_ovrdval
  VTQD_FrEDUAvailBrkRgnTqV_flg_Inproc : FVT_lib/outp/OverrideAndLimit  SystemSampleTime=-1  VariantActivationTime=update diagram  Latency=0  AutoFrameSizeCalculation=off
      link override Signal_Limit/_maxval: Value=KOUTP_FrEDUAvailBrkRgnTqV_flg_maxval
      link override Signal_Limit/_minval: Value=KOUTP_FrEDUAvailBrkRgnTqV_flg_minval
      link override Signal_Override/_ovrdflg: Value=KOUTP_FrEDUAvailBrkRgnTqV_flg_ovrdflg
      link override Signal_Override/_ovrdval: Value=KOUTP_FrEDUAvailBrkRgnTqV_flg_ovrdval
  VTQD_FrEDUAvailBrkRgnTq_Nm_Inproc : FVT_lib/outp/OverrideAndLimit  SystemSampleTime=-1  VariantActivationTime=update diagram  Latency=0  AutoFrameSizeCalculation=off
      link override Signal_Limit/_maxval: Value=KOUTP_FrEDUAvailBrkRgnTq_Nm_maxval
      link override Signal_Limit/_minval: Value=KOUTP_FrEDUAvailBrkRgnTq_Nm_minval
      link override Signal_Override/_ovrdflg: Value=KOUTP_FrEDUAvailBrkRgnTq_Nm_ovrdflg
      link override Signal_Override/_ovrdval: Value=KOUTP_FrEDUAvailBrkRgnTq_Nm_ovrdval
  VTQD_FrEDURolRgnTq_Nm_Inproc : FVT_lib/outp/OverrideAndLimit  SystemSampleTime=-1  VariantActivationTime=update diagram  Latency=0  AutoFrameSizeCalculation=off
      link override Signal_Limit/_maxval: Value=KOUTP_FrEDURolRgnTq_Nm_maxval
      link override Signal_Limit/_minval: Value=KOUTP_FrEDURolRgnTq_Nm_minval
      link override Signal_Override/_ovrdflg: Value=KOUTP_FrEDURolRgnTq_Nm_ovrdflg
      link override Signal_Override/_ovrdval: Value=KOUTP_FrEDURolRgnTq_Nm_ovrdval
  VTQD_FrEDUSpdValid_flg_Inproc : FVT_lib/outp/OverrideAndLimit  SystemSampleTime=-1  VariantActivationTime=update diagram  Latency=0  AutoFrameSizeCalculation=off
      link override Signal_Limit/_maxval: Value=KOUTP_FrEDUSpdValid_flg_maxval
      link override Signal_Limit/_minval: Value=KOUTP_FrEDUSpdValid_flg_minval
      link override Signal_Override/_ovrdflg: Value=KOUTP_FrEDUSpdValid_flg_ovrdflg
      link override Signal_Override/_ovrdval: Value=KOUTP_FrEDUSpdValid_flg_ovrdval
  VTQD_FrEDUSpd_rpm_Inproc : FVT_lib/outp/OverrideAndLimit  SystemSampleTime=-1  VariantActivationTime=update diagram  Latency=0  AutoFrameSizeCalculation=off
      link override Signal_Limit/_maxval: Value=KOUTP_FrEDUSpd_rpm_maxval
      link override Signal_Limit/_minval: Value=KOUTP_FrEDUSpd_rpm_minval
      link override Signal_Override/_ovrdflg: Value=KOUTP_FrEDUSpd_rpm_ovrdflg
      link override Signal_Override/_ovrdval: Value=KOUTP_FrEDUSpd_rpm_ovrdval
  VTQD_FrIdcMax_A_Inproc : FVT_lib/outp/OverrideAndLimit  SystemSampleTime=-1  VariantActivationTime=update diagram  Latency=0  AutoFrameSizeCalculation=off
      link override Signal_Limit/_maxval: Value=KOUTP_FrIdcMax_A_maxval
      link override Signal_Limit/_minval: Value=KOUTP_FrIdcMax_A_minval
      link override Signal_Override/_ovrdflg: Value=KOUTP_FrIdcMax_A_ovrdflg
      link override Signal_Override/_ovrdval: Value=KOUTP_FrIdcMax_A_ovrdval
  VTQD_FrIdcMin_A_Inproc : FVT_lib/outp/OverrideAndLimit  SystemSampleTime=-1  VariantActivationTime=update diagram  Latency=0  AutoFrameSizeCalculation=off
      link override Signal_Limit/_maxval: Value=KOUTP_FrIdcMin_A_maxval
      link override Signal_Limit/_minval: Value=KOUTP_FrIdcMin_A_minval
      link override Signal_Override/_ovrdflg: Value=KOUTP_FrIdcMin_A_ovrdflg
      link override Signal_Override/_ovrdval: Value=KOUTP_FrIdcMin_A_ovrdval
  VTQD_FrRgnDecrSta_flg_Inproc : FVT_lib/outp/OverrideAndLimit  SystemSampleTime=-1  VariantActivationTime=update diagram  Latency=0  AutoFrameSizeCalculation=off
      link override Signal_Limit/_maxval: Value=KOUTP_FrRgnDecrSta_flg_maxval
      link override Signal_Limit/_minval: Value=KOUTP_FrRgnDecrSta_flg_minval
      link override Signal_Override/_ovrdflg: Value=KOUTP_FrRgnDecrSta_flg_ovrdflg
      link override Signal_Override/_ovrdval: Value=KOUTP_FrRgnDecrSta_flg_ovrdval
  VTQD_FrRgnPermSta_flg_Inproc : FVT_lib/outp/OverrideAndLimit  SystemSampleTime=-1  VariantActivationTime=update diagram  Latency=0  AutoFrameSizeCalculation=off
      link override Signal_Limit/_maxval: Value=KOUTP_FrRgnPermSta_flg_maxval
      link override Signal_Limit/_minval: Value=KOUTP_FrRgnPermSta_flg_minval
      link override Signal_Override/_ovrdflg: Value=KOUTP_FrRgnPermSta_flg_ovrdflg
      link override Signal_Override/_ovrdval: Value=KOUTP_FrRgnPermSta_flg_ovrdval
  VTQD_FrUdcMax_V_Inproc : FVT_lib/outp/OverrideAndLimit  SystemSampleTime=-1  VariantActivationTime=update diagram  Latency=0  AutoFrameSizeCalculation=off
      link override Signal_Limit/_maxval: Value=KOUTP_FrUdcMax_V_maxval
      link override Signal_Limit/_minval: Value=KOUTP_FrUdcMax_V_minval
      link override Signal_Override/_ovrdflg: Value=KOUTP_FrUdcMax_V_ovrdflg
      link override Signal_Override/_ovrdval: Value=KOUTP_FrUdcMax_V_ovrdval
  VTQD_FrUdcMin_V_Inproc : FVT_lib/outp/OverrideAndLimit  SystemSampleTime=-1  VariantActivationTime=update diagram  Latency=0  AutoFrameSizeCalculation=off
      link override Signal_Limit/_maxval: Value=KOUTP_FrUdcMin_V_maxval
      link override Signal_Limit/_minval: Value=KOUTP_FrUdcMin_V_minval
      link override Signal_Override/_ovrdflg: Value=KOUTP_FrUdcMin_V_ovrdflg
      link override Signal_Override/_ovrdval: Value=KOUTP_FrUdcMin_V_ovrdval
  VTQD_IVIPwrLockSta_enum_Inproc : FVT_lib/outp/OverrideAndLimit  SystemSampleTime=-1  VariantActivationTime=update diagram  Latency=0  AutoFrameSizeCalculation=off
      link override Signal_Limit/_maxval: Value=KOUTP_IVIPwrLockSta_enum_maxval
      link override Signal_Limit/_minval: Value=KOUTP_IVIPwrLockSta_enum_minval
      link override Signal_Override/_ovrdflg: Value=KOUTP_IVIPwrLockSta_enum_ovrdflg
      link override Signal_Override/_ovrdval: Value=KOUTP_IVIPwrLockSta_enum_ovrdval
  VTQD_MaxWhlSlideRate_pct_Inproc : FVT_lib/outp/OverrideAndLimit  SystemSampleTime=-1  VariantActivationTime=update diagram  Latency=0  AutoFrameSizeCalculation=off
      link override Signal_Limit/_maxval: Value=KOUTP_MaxWhlSlideRate_pct_maxval
      link override Signal_Limit/_minval: Value=KOUTP_MaxWhlSlideRate_pct_minval
      link override Signal_Override/_ovrdflg: Value=KOUTP_MaxWhlSlideRate_pct_ovrdflg
      link override Signal_Override/_ovrdval: Value=KOUTP_MaxWhlSlideRate_pct_ovrdval
  VTQD_OPDHoldLamp_flg_Inproc : FVT_lib/outp/OverrideAndLimit  SystemSampleTime=-1  VariantActivationTime=update diagram  Latency=0  AutoFrameSizeCalculation=off
      link override Signal_Limit/_maxval: Value=KOUTP_OPDHoldLamp_flg_maxval
      link override Signal_Limit/_minval: Value=KOUTP_OPDHoldLamp_flg_minval
      link override Signal_Override/_ovrdflg: Value=KOUTP_OPDHoldLamp_flg_ovrdflg
      link override Signal_Override/_ovrdval: Value=KOUTP_OPDHoldLamp_flg_ovrdval
  VTQD_PButtonSta_enum_Inproc : FVT_lib/outp/OverrideAndLimit  SystemSampleTime=-1  VariantActivationTime=update diagram  Latency=0  AutoFrameSizeCalculation=off
      link override Signal_Limit/_maxval: Value=KOUTP_PButtonSta_enum_maxval
      link override Signal_Limit/_minval: Value=KOUTP_PButtonSta_enum_minval
      link override Signal_Override/_ovrdflg: Value=KOUTP_PButtonSta_enum_ovrdflg
      link override Signal_Override/_ovrdval: Value=KOUTP_PButtonSta_enum_ovrdval
  VTQD_PTCSPermSta_flg_Inproc : FVT_lib/outp/OverrideAndLimit  SystemSampleTime=-1  VariantActivationTime=update diagram  Latency=0  AutoFrameSizeCalculation=off
      link override Signal_Limit/_maxval: Value=KOUTP_PTCSPermSta_flg_maxval
      link override Signal_Limit/_minval: Value=KOUTP_PTCSPermSta_flg_minval
      link override Signal_Override/_ovrdflg: Value=KOUTP_PTCSPermSta_flg_ovrdflg
      link override Signal_Override/_ovrdval: Value=KOUTP_PTCSPermSta_flg_ovrdval
  VTQD_ParkRequest_flg_Inproc : FVT_lib/outp/OverrideAndLimit  SystemSampleTime=-1  VariantActivationTime=update diagram  Latency=0  AutoFrameSizeCalculation=off
      link override Signal_Limit/_maxval: Value=KOUTP_ParkRequest_flg_maxval
      link override Signal_Limit/_minval: Value=KOUTP_ParkRequest_flg_minval
      link override Signal_Override/_ovrdflg: Value=KOUTP_ParkRequest_flg_ovrdflg
      link override Signal_Override/_ovrdval: Value=KOUTP_ParkRequest_flg_ovrdval
  VTQD_RDCActive_enum_Inproc : FVT_lib/outp/OverrideAndLimit  SystemSampleTime=-1  VariantActivationTime=update diagram  Latency=0  AutoFrameSizeCalculation=off
      link override Signal_Limit/_maxval: Value=KOUTP_RDCActive_enum_maxval
      link override Signal_Limit/_minval: Value=KOUTP_RDCActive_enum_minval
      link override Signal_Override/_ovrdflg: Value=KOUTP_RDCActive_enum_ovrdflg
      link override Signal_Override/_ovrdval: Value=KOUTP_RDCActive_enum_ovrdval
  VTQD_ReBrakeLPReq_flg_Inproc : FVT_lib/outp/OverrideAndLimit  SystemSampleTime=-1  VariantActivationTime=update diagram  Latency=0  AutoFrameSizeCalculation=off
      link override Signal_Limit/_maxval: Value=KOUTP_ReBrakeLPReq_flg_maxval
      link override Signal_Limit/_minval: Value=KOUTP_ReBrakeLPReq_flg_minval
      link override Signal_Override/_ovrdflg: Value=KOUTP_ReBrakeLPReq_flg_ovrdflg
      link override Signal_Override/_ovrdval: Value=KOUTP_ReBrakeLPReq_flg_ovrdval
  VTQD_RegenLimIndSta_flg_Inproc : FVT_lib/outp/OverrideAndLimit  SystemSampleTime=-1  VariantActivationTime=update diagram  Latency=0  AutoFrameSizeCalculation=off
      link override Signal_Limit/_maxval: Value=KOUTP_RegenLimIndSta_flg_maxval
      link override Signal_Limit/_minval: Value=KOUTP_RegenLimIndSta_flg_minval
      link override Signal_Override/_ovrdflg: Value=KOUTP_RegenLimIndSta_flg_ovrdflg
      link override Signal_Override/_ovrdval: Value=KOUTP_RegenLimIndSta_flg_ovrdval
  VTQD_RegenTqLimitEn_flg_Inproc : FVT_lib/outp/OverrideAndLimit  SystemSampleTime=-1  VariantActivationTime=update diagram  Latency=0  AutoFrameSizeCalculation=off
      link override Signal_Limit/_maxval: Value=KOUTP_RegenTqLimitEn_flg_maxval
      link override Signal_Limit/_minval: Value=KOUTP_RegenTqLimitEn_flg_minval
      link override Signal_Override/_ovrdflg: Value=KOUTP_RegenTqLimitEn_flg_ovrdflg
      link override Signal_Override/_ovrdval: Value=KOUTP_RegenTqLimitEn_flg_ovrdval
  VTQD_RgnAbnorSta_flg_Inproc : FVT_lib/outp/OverrideAndLimit  SystemSampleTime=-1  VariantActivationTime=update diagram  Latency=0  AutoFrameSizeCalculation=off
      link override Signal_Limit/_maxval: Value=KOUTP_RgnAbnorSta_flg_maxval
      link override Signal_Limit/_minval: Value=KOUTP_RgnAbnorSta_flg_minval
      link override Signal_Override/_ovrdflg: Value=KOUTP_RgnAbnorSta_flg_ovrdflg
      link override Signal_Override/_ovrdval: Value=KOUTP_RgnAbnorSta_flg_ovrdval
  VTQD_RrActvDmpDisabReq_flg_Inproc : FVT_lib/outp/OverrideAndLimit  SystemSampleTime=-1  VariantActivationTime=update diagram  Latency=0  AutoFrameSizeCalculation=off
      link override Signal_Limit/_maxval: Value=KOUTP_RrActvDmpDisabReq_flg_maxval
      link override Signal_Limit/_minval: Value=KOUTP_RrActvDmpDisabReq_flg_minval
      link override Signal_Override/_ovrdflg: Value=KOUTP_RrActvDmpDisabReq_flg_ovrdflg
      link override Signal_Override/_ovrdval: Value=KOUTP_RrActvDmpDisabReq_flg_ovrdval
  VTQD_RrEDUActTq_Nm_Inproc : FVT_lib/outp/OverrideAndLimit  SystemSampleTime=-1  VariantActivationTime=update diagram  Latency=0  AutoFrameSizeCalculation=off
      link override Signal_Limit/_maxval: Value=KOUTP_RrEDUActTq_Nm_maxval
      link override Signal_Limit/_minval: Value=KOUTP_RrEDUActTq_Nm_minval
      link override Signal_Override/_ovrdflg: Value=KOUTP_RrEDUActTq_Nm_ovrdflg
      link override Signal_Override/_ovrdval: Value=KOUTP_RrEDUActTq_Nm_ovrdval
  VTQD_RrEDUAvailBrkRgnTqV_flg_Inproc : FVT_lib/outp/OverrideAndLimit  SystemSampleTime=-1  VariantActivationTime=update diagram  Latency=0  AutoFrameSizeCalculation=off
      link override Signal_Limit/_maxval: Value=KOUTP_RrEDUAvailBrkRgnTqV_flg_maxval
      link override Signal_Limit/_minval: Value=KOUTP_RrEDUAvailBrkRgnTqV_flg_minval
      link override Signal_Override/_ovrdflg: Value=KOUTP_RrEDUAvailBrkRgnTqV_flg_ovrdflg
      link override Signal_Override/_ovrdval: Value=KOUTP_RrEDUAvailBrkRgnTqV_flg_ovrdval
  VTQD_RrEDUAvailBrkRgnTq_Nm_Inproc : FVT_lib/outp/OverrideAndLimit  SystemSampleTime=-1  VariantActivationTime=update diagram  Latency=0  AutoFrameSizeCalculation=off
      link override Signal_Limit/_maxval: Value=KOUTP_RrEDUAvailBrkRgnTq_Nm_maxval
      link override Signal_Limit/_minval: Value=KOUTP_RrEDUAvailBrkRgnTq_Nm_minval
      link override Signal_Override/_ovrdflg: Value=KOUTP_RrEDUAvailBrkRgnTq_Nm_ovrdflg
      link override Signal_Override/_ovrdval: Value=KOUTP_RrEDUAvailBrkRgnTq_Nm_ovrdval
  VTQD_RrEDURolRgnTq_Nm_Inproc : FVT_lib/outp/OverrideAndLimit  SystemSampleTime=-1  VariantActivationTime=update diagram  Latency=0  AutoFrameSizeCalculation=off
      link override Signal_Limit/_maxval: Value=KOUTP_RrEDURolRgnTq_Nm_maxval
      link override Signal_Limit/_minval: Value=KOUTP_RrEDURolRgnTq_Nm_minval
      link override Signal_Override/_ovrdflg: Value=KOUTP_RrEDURolRgnTq_Nm_ovrdflg
      link override Signal_Override/_ovrdval: Value=KOUTP_RrEDURolRgnTq_Nm_ovrdval
  VTQD_RrEDUSpdValid_flg_Inproc : FVT_lib/outp/OverrideAndLimit  SystemSampleTime=-1  VariantActivationTime=update diagram  Latency=0  AutoFrameSizeCalculation=off
      link override Signal_Limit/_maxval: Value=KOUTP_RrEDUSpdValid_flg_maxval
      link override Signal_Limit/_minval: Value=KOUTP_RrEDUSpdValid_flg_minval
      link override Signal_Override/_ovrdflg: Value=KOUTP_RrEDUSpdValid_flg_ovrdflg
      link override Signal_Override/_ovrdval: Value=KOUTP_RrEDUSpdValid_flg_ovrdval
  VTQD_RrEDUSpd_rpm_Inproc : FVT_lib/outp/OverrideAndLimit  SystemSampleTime=-1  VariantActivationTime=update diagram  Latency=0  AutoFrameSizeCalculation=off
      link override Signal_Limit/_maxval: Value=KOUTP_RrEDUSpd_rpm_maxval
      link override Signal_Limit/_minval: Value=KOUTP_RrEDUSpd_rpm_minval
      link override Signal_Override/_ovrdflg: Value=KOUTP_RrEDUSpd_rpm_ovrdflg
      link override Signal_Override/_ovrdval: Value=KOUTP_RrEDUSpd_rpm_ovrdval
  VTQD_RrIdcMax_A_Inproc : FVT_lib/outp/OverrideAndLimit  SystemSampleTime=-1  VariantActivationTime=update diagram  Latency=0  AutoFrameSizeCalculation=off
      link override Signal_Limit/_maxval: Value=KOUTP_RrIdcMax_A_maxval
      link override Signal_Limit/_minval: Value=KOUTP_RrIdcMax_A_minval
      link override Signal_Override/_ovrdflg: Value=KOUTP_RrIdcMax_A_ovrdflg
      link override Signal_Override/_ovrdval: Value=KOUTP_RrIdcMax_A_ovrdval
  VTQD_RrIdcMin_A_Inproc : FVT_lib/outp/OverrideAndLimit  SystemSampleTime=-1  VariantActivationTime=update diagram  Latency=0  AutoFrameSizeCalculation=off
      link override Signal_Limit/_maxval: Value=KOUTP_RrIdcMin_A_maxval
      link override Signal_Limit/_minval: Value=KOUTP_RrIdcMin_A_minval
      link override Signal_Override/_ovrdflg: Value=KOUTP_RrIdcMin_A_ovrdflg
      link override Signal_Override/_ovrdval: Value=KOUTP_RrIdcMin_A_ovrdval
  VTQD_RrRgnDecrSta_flg_Inproc : FVT_lib/outp/OverrideAndLimit  SystemSampleTime=-1  VariantActivationTime=update diagram  Latency=0  AutoFrameSizeCalculation=off
      link override Signal_Limit/_maxval: Value=KOUTP_RrRgnDecrSta_flg_maxval
      link override Signal_Limit/_minval: Value=KOUTP_RrRgnDecrSta_flg_minval
      link override Signal_Override/_ovrdflg: Value=KOUTP_RrRgnDecrSta_flg_ovrdflg
      link override Signal_Override/_ovrdval: Value=KOUTP_RrRgnDecrSta_flg_ovrdval
  VTQD_RrRgnPermSta_flg_Inproc : FVT_lib/outp/OverrideAndLimit  SystemSampleTime=-1  VariantActivationTime=update diagram  Latency=0  AutoFrameSizeCalculation=off
      link override Signal_Limit/_maxval: Value=KOUTP_RrRgnPermSta_flg_maxval
      link override Signal_Limit/_minval: Value=KOUTP_RrRgnPermSta_flg_minval
      link override Signal_Override/_ovrdflg: Value=KOUTP_RrRgnPermSta_flg_ovrdflg
      link override Signal_Override/_ovrdval: Value=KOUTP_RrRgnPermSta_flg_ovrdval
  VTQD_RrUdcMax_V_Inproc : FVT_lib/outp/OverrideAndLimit  SystemSampleTime=-1  VariantActivationTime=update diagram  Latency=0  AutoFrameSizeCalculation=off
      link override Signal_Limit/_maxval: Value=KOUTP_RrUdcMax_V_maxval
      link override Signal_Limit/_minval: Value=KOUTP_RrUdcMax_V_minval
      link override Signal_Override/_ovrdflg: Value=KOUTP_RrUdcMax_V_ovrdflg
      link override Signal_Override/_ovrdval: Value=KOUTP_RrUdcMax_V_ovrdval
  VTQD_RrUdcMin_V_Inproc : FVT_lib/outp/OverrideAndLimit  SystemSampleTime=-1  VariantActivationTime=update diagram  Latency=0  AutoFrameSizeCalculation=off
      link override Signal_Limit/_maxval: Value=KOUTP_RrUdcMin_V_maxval
      link override Signal_Limit/_minval: Value=KOUTP_RrUdcMin_V_minval
      link override Signal_Override/_ovrdflg: Value=KOUTP_RrUdcMin_V_ovrdflg
      link override Signal_Override/_ovrdval: Value=KOUTP_RrUdcMin_V_ovrdval
